simulink library "ammclib_bam_S32K3xx"  (R2016a)
settings: Solver=VariableStepAuto  SolverMode=SingleTasking  StartTime=0.0  StopTime=10.0  RelTol=1e-3
undefined symbols (not defined in the file or in its folder): a1, a2, ADCMaxError, autoCalcEn, b0, b1, b2, cfg, dgain, escale, f16A1, f16A2, f16ADCMaxError, f16B0, f16B1, f16B2, f16C1, f16CC1sc, f16CC1sc_D, f16CC1sc_Q, f16CC2sc, f16CC2sc_D, f16CC2sc_Q, f16DerivGain, f16EGain, f16FiltCoef, f16HystOff, f16HystOn, f16IGain, f16IntegGain, f16IntegGain_D, f16IntegGain_Q, f16IntegGainQ, f16Kd, f16KLs, f16Kq, f16KRs, f16Limit, f16LowerLimit, f16LowerLimit_D, f16LowerLimit_Q, f16LowerLimitQ, f16ModIndex, f16OutValOff, f16OutValOn, f16PropGain, f16PropGain_D, f16PropGain_Q, f16PropGainQ, f16RampDown, f16RampUp, f16UGain, f16UpperLimit, f16UpperLimit_D, f16UpperLimit_Q, f16UpperLimitQ, f16WIGain, f32A1, f32A2, f32ADCMaxError ... (+180)
(part 35 of 50)

== system ammclib_bam_S32K3xx/GFLIB/F32 ==
  GFLIB_Acos_F32 : Subsystem  TreatAsAtomicUnit=on  mask(GFLIB_Acos_F32){}
      mask help: Inverse cosine function in 32-bit fixed-point fractional implementation. Refer to the AMMCLIB User's Guide for further details.
      mask init: same as ammclib_bam_S32K3xx/GDFLIB/F16/GDFLIB_FilterFIR_F16
      settings: RTWSystemCode=Inline
      mask Help: web([fileparts(which('ammclib_bam_S32K3xx.slx')) '/../doc/S32K3XXMCLUG.pdf'], '-browser')
      mask Display: pos = get_param(gcb, 'Position');width = pos(3) - pos(1); height = pos(4) - pos(2);tX=width/2;tY=height - 8;color('black');text(tX,tY, 'GFLIB_Acos_F32', 'horizontalAlignment', 'center');
  GFLIB_Asin_F32 : Subsystem  TreatAsAtomicUnit=on  mask(GFLIB_Asin_F32){}
      mask help: Inverse sine function in 32-bit fixed-point fractional implementation. Refer to the AMMCLIB User's Guide for further details.
      mask init: same as ammclib_bam_S32K3xx/GDFLIB/F16/GDFLIB_FilterFIR_F16
      settings: RTWSystemCode=Inline
      mask Help: web([fileparts(which('ammclib_bam_S32K3xx.slx')) '/../doc/S32K3XXMCLUG.pdf'], '-browser')
      mask Display: pos = get_param(gcb, 'Position');width = pos(3) - pos(1); height = pos(4) - pos(2);tX=width/2;tY=height - 8;color('black');text(tX,tY, 'GFLIB_Asin_F32', 'horizontalAlignment', 'center');
  GFLIB_AtanYXShifted_F32 : Subsystem  TreatAsAtomicUnit=on  mask(GFLIB_AtanYXShifted_F32){}
      mask help: Shifted arctangent of two arguments Y/X in 32-bit fixed-point fractional implementation. Refer to the AMMCLIB User's Guide for further details.
      mask init: same as ammclib_bam_S32K3xx/GDFLIB/F16/GDFLIB_FilterFIR_F16
      settings: RTWSystemCode=Inline
      mask Help: web([fileparts(which('ammclib_bam_S32K3xx.slx')) '/../doc/S32K3XXMCLUG.pdf'], '-browser')
      mask Display: pos = get_param(gcb, 'Position');width = pos(3) - pos(1); height = pos(4) - pos(2);tX=width/2;tY=height - 8;color('black');text(tX,tY, 'GFLIB_AtanYXShifted_F32', 'horizontalAlignment', 'center');
  GFLIB_AtanYX_F32 : Subsystem  TreatAsAtomicUnit=on  mask(GFLIB_AtanYX_F32){}
      mask help: Arctangent of two arguments Y/X in 32-bit fixed-point fractional implementation. Refer to the AMMCLIB User's Guide for further details.
      mask init: same as ammclib_bam_S32K3xx/GDFLIB/F16/GDFLIB_FilterFIR_F16
      settings: RTWSystemCode=Inline
      mask Help: web([fileparts(which('ammclib_bam_S32K3xx.slx')) '/../doc/S32K3XXMCLUG.pdf'], '-browser')
      mask Display: pos = get_param(gcb, 'Position');width = pos(3) - pos(1); height = pos(4) - pos(2);tX=width/2;tY=height - 8;color('black');text(tX,tY, 'GFLIB_AtanYX_F32', 'horizontalAlignment', 'center');
  GFLIB_Atan_F32 : Subsystem  TreatAsAtomicUnit=on  mask(GFLIB_Atan_F32){}
      mask help: Inverse tangent function in 32-bit fixed-point fractional implementation. Refer to the AMMCLIB User's Guide for further details.
      mask init: same as ammclib_bam_S32K3xx/GDFLIB/F16/GDFLIB_FilterFIR_F16
      settings: RTWSystemCode=Inline
      mask Help: web([fileparts(which('ammclib_bam_S32K3xx.slx')) '/../doc/S32K3XXMCLUG.pdf'], '-browser')
      mask Display: pos = get_param(gcb, 'Position');width = pos(3) - pos(1); height = pos(4) - pos(2);tX=width/2;tY=height - 8;color('black');text(tX,tY, 'GFLIB_Atan_F32', 'horizontalAlignment', 'center');
  GFLIB_ControllerPIDpAW_F32 : Subsystem  StartFcn=|  TreatAsAtomicUnit=on  mask(GFLIB_ControllerPIDpAW_F32){showStates=Hide (faster execution), resetStatesEnable=Pre-set according to the first set of inputs after reset, SampleTime=-1, pgain=5, igain=0.5, dgain=0.01, filtCoef=10, lowerLimit=-10, upperLimit=9.999999995343387, inscale=10, outscale=10, autoCalcEn=on, f32PropGain=0, f32IntegGain=0, f32DerivGain=0, f32FiltCoef=0, s16PropGainShift=0, s16IntegGainShift=0, s16DerivGainShift=0, f32LowerLimit=0, f32UpperLimit=0, SampleTime_1=NaN}
      | ts=get_param(gcb,'CompiledSampleTime');
      | if iscell(ts)
      |   ts=ts{1};
      |   if iscell(ts)
      |     ts=ts{1};
      |   end
      | end
      | ts=ts(1);
      | set_param(gcb,'SampleTime_1',num2str(ts));
      | p=Simulink.Mask.get(gcb);
      | hintText=p.getDialogControl('timeHint');
      | SampleTime=Simulink.data.evalinGlobal(bdroot,get_param(gcb,'SampleTime'));
      | p=Simulink.Mask.get(gcb);
      | autoCalcEn=get_param(gcb,'autoCalcEn');
      | if strcmp(autoCalcEn,'on')
      |   if SampleTime==-1
      |     hintText.Prompt='Caution: Implementation parameters depend on inherited sample time. Make sure that the sample time of the block''s inputs corresponds to the sampling period in the target application.';
      |   else
      |     hintText.Prompt='Caution: Implementation parameters depend on the sample time. Make sure that the simulation time step corresponds to the sampling period in the target application.';
      |   end
      |   SampleTime=ts;
      |   f32PropGain_bkup=get_param(gcb,'f32PropGain');
      |   f32IntegGain_bkup=get_param(gcb,'f32IntegGain');
      |   f32DerivGain_bkup=get_param(gcb,'f32DerivGain');
      |   f32FiltCoef_bkup=get_param(gcb,'f32FiltCoef');
      |   s16PropGainShift_bkup=get_param(gcb,'s16PropGainShift');
      |   s16IntegGainShift_bkup=get_param(gcb,'s16IntegGainShift');
      |   s16DerivGainShift_bkup=get_param(gcb,'s16DerivGainShift');
      |   f32LowerLimit_bkup=get_param(gcb,'f32LowerLimit');
      |   f32UpperLimit_bkup=get_param(gcb,'f32UpperLimit');
      |   pgain=Simulink.data.evalinGlobal(bdroot,get_param(gcb,'pgain'));
      |   igain=Simulink.data.evalinGlobal(bdroot,get_param(gcb,'igain'));
      |   dgain=Simulink.data.evalinGlobal(bdroot,get_param(gcb,'dgain'));
      |   filtCoef=Simulink.data.evalinGlobal(bdroot,get_param(gcb,'filtCoef'));
      |   lowerLimit=Simulink.data.evalinGlobal(bdroot,get_param(gcb,'lowerLimit'));
      |   upperLimit=Simulink.data.evalinGlobal(bdroot,get_param(gcb,'upperLimit'));
      |   inscale=Simulink.data.evalinGlobal(bdroot,get_param(gcb,'inscale'));
      |   outscale=Simulink.data.evalinGlobal(bdroot,get_param(gcb,'outscale'));
      |   if (upperLimit<=lowerLimit)
      |     warning('UpperLimit should be greater than LowerLimit.');
      |   end
      |   if (inscale<=0)
      |     warning('E_max must be positive.');
      |   end
      |   if (outscale<=0)
      |     warning('U_max must be positive.');
      |   end
      |   kpf=pgain*inscale/outscale;
      |   s16PropGainShift=ceil(log2(abs(kpf)));
      |   if s16PropGainShift<-31
      |     s16PropGainShift=-31;
      |   end
      |   if s16PropGainShift>31
      |     s16PropGainShift=31;
      |     warning(['Parameter s16PropGainShift of ' gcb ' exceeds the fixed-point range.']);
      |   end
      |   f32PropGain=round(kpf*2^(-s16PropGainShift)*2^31);
      |   if f32PropGain>2^31-1
      |     f32PropGain=2^31-1;
      |     warning(['Parameter f32PropGain of ' gcb ' exceeds the fixed-point range.']);
      |   end
      |   if f32PropGain<-2^31
      |     f32PropGain=-2^31;
      |     warning(['Parameter f32PropGain of ' gcb ' exceeds the fixed-point range.']);
      |   end
      |   kif=igain*SampleTime*0.5*inscale/outscale;
      |   s16IntegGainShift=ceil(log2(abs(kif)));
      |   if s16IntegGainShift<-31
      |     s16IntegGainShift=-31;
      |   end
      |   if s16IntegGainShift>31
      |     s16IntegGainShift=31;
      |     warning(['Parameter s16IntegGainShift of ' gcb ' exceeds the fixed-point range.']);
      |   end
      |   f32IntegGain=round(kif*2^(-s16IntegGainShift)*2^31);
      |   if f32IntegGain>2^31-1
      |     f32IntegGain=2^31-1;
      |     warning(['Parameter f32IntegGain of ' gcb ' exceeds the fixed-point range.']);
      |   end
      |   if f32IntegGain<-2^31
      |     f32IntegGain=-2^31;
      |     warning(['Parameter f32IntegGain of ' gcb ' exceeds the fixed-point range.']);
      |   end
      |   upperLimitf=upperLimit/outscale;
      |   lowerLimitf=lowerLimit/outscale;
      |   f32UpperLimit=round(upperLimitf*2^31);
      |   if f32UpperLimit>2^31-1
      |     f32UpperLimit=2^31-1;
      |     warning(['Parameter f32UpperLimit of ' gcb ' exceeds the fixed-point range.']);
      |   end
      |   if f32UpperLimit<-2^31
      |     f32UpperLimit=-2^31;
      |     warning(['Parameter f32UpperLimit of ' gcb ' exceeds the fixed-point range.']);
      |   end
      |   f32LowerLimit=round(lowerLimitf*2^31);
      |   if f32LowerLimit>2^31-1
      |     f32LowerLimit=2^31-1;
      |     warning(['Parameter f32LowerLimit of ' gcb ' exceeds the fixed-point range.']);
      |   end
      |   if f32LowerLimit<-2^31
      |     f32LowerLimit=-2^31;
      |     warning(['Parameter f32LowerLimit of ' gcb ' exceeds the fixed-point range.']);
      |   end
      |   exparg=-SampleTime*filtCoef;
      |   expconst=exp(exparg);
      |   f32FiltCoef=round(expconst*2^31);
      |   if f32FiltCoef>2^31-1
      |     f32FiltCoef=2^31-1;
      |     warning(['Parameter f32FiltCoef of ' gcb ' exceeds the fixed-point range.']);
      |   end
      |   if f32FiltCoef<-2^31
      |     f32FiltCoef=-2^31;
      |     warning(['Parameter f32FiltCoef of ' gcb ' exceeds the fixed-point range.']);
      |   end
      |   kdf=dgain/SampleTime*(1 - expconst)*inscale/outscale;
      |   s16DerivGainShift=ceil(log2(abs(kpf)));
      |   if s16DerivGainShift<-31
      |     s16DerivGainShift=-31;
      |   end
      |   if s16DerivGainShift>31
      |     s16DerivGainShift=31;
      |     warning(['Parameter s16DerivGainShift of ' gcb ' exceeds the fixed-point range.']);
      |   end
      |   f32DerivGain=round(kpf*2^(-s16DerivGainShift)*2^31);
      |   if f32DerivGain>2^31-1
      |     f32DerivGain=2^31-1;
      |     warning(['Parameter f32DerivGain of ' gcb ' exceeds the fixed-point range.']);
      |   end
      |   if f32DerivGain<-2^31
      |     f32DerivGain=-2^31;
      |     warning(['Parameter f32DerivGain of ' gcb ' exceeds the fixed-point range.']);
      |   end
      |   if isnan(f32PropGain)
      |     if ~strcmp(f32PropGain_bkup,'0')
      |       set_param(gcb,'f32PropGain','0');
      |     end
      |   else
      |     tmps=num2str(f32PropGain);
      |     if ~strcmp(f32PropGain_bkup,tmps)
      |       set_param(gcb,'f32PropGain',tmps);
      |     end
      |   end
      |   if isnan(f32IntegGain)
      |     if ~strcmp(f32IntegGain_bkup,'0')
      |       set_param(gcb,'f32IntegGain','0');
      |     end
      |   else
      |     tmps=num2str(f32IntegGain);
      |     if ~strcmp(f32IntegGain_bkup,tmps)
      |       set_param(gcb,'f32IntegGain',tmps);
      |     end
      |   end
      |   if isnan(f32DerivGain)
      |     if ~strcmp(f32DerivGain_bkup,'0')
      |       set_param(gcb,'f32DerivGain','0');
      |     end
      |   else
      |     tmps=num2str(f32DerivGain);
      |     if ~strcmp(f32DerivGain_bkup,tmps)
      |       set_param(gcb,'f32DerivGain',tmps);
      |     end
      |   end
      |   if isnan(f32FiltCoef)
      |     if ~strcmp(f32FiltCoef_bkup,'0')
      |       set_param(gcb,'f32FiltCoef','0');
      |     end
      |   else
      |     tmps=num2str(f32FiltCoef);
      |     if ~strcmp(f32FiltCoef_bkup,tmps)
      |       set_param(gcb,'f32FiltCoef',tmps);
      |     end
      |   end
      |   if isnan(s16PropGainShift)
      |     if ~strcmp(s16PropGainShift_bkup,'0')
      |       set_param(gcb,'s16PropGainShift','0');
      |     end
      |   else
      |     tmps=num2str(s16PropGainShift);
      |     if ~strcmp(s16PropGainShift_bkup,tmps)
      |       set_param(gcb,'s16PropGainShift',tmps);
      |     end
      |   end
      |   if isnan(s16IntegGainShift)
      |     if ~strcmp(s16IntegGainShift_bkup,'0')
      |       set_param(gcb,'s16IntegGainShift','0');
      |     end
      |   else
      |     tmps=num2str(s16IntegGainShift);
      |     if ~strcmp(s16IntegGainShift_bkup,tmps)
      |       set_param(gcb,'s16IntegGainShift',tmps);
      |     end
      |   end
      |   if isnan(s16DerivGainShift)
      |     if ~strcmp(s16DerivGainShift_bkup,'0')
      |       set_param(gcb,'s16DerivGainShift','0');
      |     end
      |   else
      |     tmps=num2str(s16DerivGainShift);
      |     if ~strcmp(s16DerivGainShift_bkup,tmps)
      |       set_param(gcb,'s16DerivGainShift',tmps);
      |     end
      |   end
      |   if isnan(f32LowerLimit)
      |     if ~strcmp(f32LowerLimit_bkup,'0')
      |       set_param(gcb,'f32LowerLimit','0');
      |     end
      |   else
      |     tmps=num2str(f32LowerLimit);
      |     if ~strcmp(f32LowerLimit_bkup,tmps)
      |       set_param(gcb,'f32LowerLimit',tmps);
      |     end
      |   end
      |   if isnan(f32UpperLimit)
      |     if ~strcmp(f32UpperLimit_bkup,'0')
      |       set_param(gcb,'f32UpperLimit','0');
      |     end
      |   else
      |     tmps=num2str(f32UpperLimit);
      |     if ~strcmp(f32UpperLimit_bkup,tmps)
      |       set_param(gcb,'f32UpperLimit',tmps);
      |     end
      |   end
      | end
      mask prompts: showStates "Show internal states:"; resetStatesEnable "Internal state after reset:"; SampleTime "Sample time (-1 for inherited):"; pgain "Proportional gain (P):"; igain "Integral gain (I):"; dgain "Derivative gain (D):"; filtCoef "Derivative gain limit N (usually 3 to 20):"; lowerLimit "Controller lower limit:"; upperLimit "Controller upper limit:"; inscale "E_max (input scale):"; outscale "U_max (output scale):"; autoCalcEn "Calculate implementation parameters from physical parameters"; f32PropGain "f32PropGain (Proportional gain):"; f32IntegGain "f32IntegGain (Integral gain):"; f32DerivGain "f32DerivGain (Derivative gain):"; f32FiltCoef "f32FiltCoef (Derivative term filter coefficient):"; s16PropGainShift "s16PropGainShift (Proportional gain shift):"; s16IntegGainShift "s16IntegGainShift (Integral gain shift):"; s16DerivGainShift "s16DerivGainShift (Derivative gain shift):"; f32LowerLimit "f32LowerLimit (Lower limit of the controller):"; f32UpperLimit "f32UpperLimit (Upper limit of the controller):"; SampleTime_1 "Discrete sample time:"
      mask help: Parallel form of a discrete-time PID controller with anti-windup in 32-bit fixed-point fractional implementation. This block supports re-initialization of the internal state during simulation. If the block is reset, the controller's output will be aligned with the input f32ControllerPIDpAWOut_preset. Refer to the AMMCLIB User's Guide for further details.
      mask init:
      | ddName = get_param(bdroot,'DataDictionary');
      | if length(ddName)==0
      |   set_param(bdroot,'DataDictionary','ammclib_types.sldd');
      | else
      |   dd = Simulink.data.dictionary.open(ddName);
      |   data = getSection(dd,'Design Data');
      |   if ~exist(data,'SWLIBS_2Syst_F16')
      |     addDataSource(dd,'ammclib_types.sldd');
      |     saveChanges(dd);
      |   end
      | end
      | 
      | if showStates == 1
      |   % hidden state variables
      |   if strcmp(get_param([gcb '/f32PropGain'], 'BlockType'), 'Inport')
      |     posblk = get_param(gcb, 'Position');
      | 
      |     pos = get_param([gcb, '/f32PropGain'], 'Position');
      |     orient = get_param([gcb, '/f32PropGain'], 'Orientation');
      |     delete_block([gcb, '/f32PropGain']);
      |     add_block('built-in/Ground', [gcb, '/f32PropGain'], 'Position', pos, 'Orientation', orient);
      | 
      |     pos = get_param([gcb, '/f32IntegGain'], 'Position');
      |     orient = get_param([gcb, '/f32IntegGain'], 'Orientation');
      |     delete_block([gcb, '/f32IntegGain']);
      |     add_block('built-in/Ground', [gcb, '/f32IntegGain'], 'Position', pos, 'Orientation', orient);
      | 
      |     pos = get_param([gcb, '/f32DerivGain'], 'Position');
      |     orient = get_param([gcb, '/f32DerivGain'], 'Orientation');
      |     delete_block([gcb, '/f32DerivGain']);
      |     add_block('built-in/Ground', [gcb, '/f32DerivGain'], 'Position', pos, 'Orientation', orient);
      | 
      |     pos = get_param([gcb, '/f32FiltCoef'], 'Position');
      |     orient = get_param([gcb, '/f32FiltCoef'], 'Orientation');
      |     delete_block([gcb, '/f32FiltCoef']);
      |     add_block('built-in/Ground', [gcb, '/f32FiltCoef'], 'Position', pos, 'Orientation', orient);
      | 
      |     pos = get_param([gcb, '/s16PropGainShift'], 'Position');
      |     orient = get_param([gcb, '/s16PropGainShift'], 'Orientation');
      |     delete_block([gcb, '/s16PropGainShift']);
      |     add_block('built-in/Ground', [gcb, '/s16PropGainShift'], 'Position', pos, 'Orientation', orient);
      | 
      |     pos = get_param([gcb, '/s16IntegGainShift'], 'Position');
      |     orient = get_param([gcb, '/s16IntegGainShift'], 'Orientation');
      |     delete_block([gcb, '/s16IntegGainShift']);
      |     add_block('built-in/Ground', [gcb, '/s16IntegGainShift'], 'Position', pos, 'Orientation', orient);
      | 
      |     pos = get_param([gcb, '/s16DerivGainShift'], 'Position');
      |     orient = get_param([gcb, '/s16DerivGainShift'], 'Orientation');
      |     delete_block([gcb, '/s16DerivGainShift']);
      |     add_block('built-in/Ground', [gcb, '/s16DerivGainShift'], 'Position', pos, 'Orientation', orient);
      | 
      |     pos = get_param([gcb, '/f32LowerLimit'], 'Position');
      |     orient = get_param([gcb, '/f32LowerLimit'], 'Orientation');
      |     delete_block([gcb, '/f32LowerLimit']);
      |     add_block('built-in/Ground', [gcb, '/f32LowerLimit'], 'Position', pos, 'Orientation', orient);
      | 
      |     pos = get_param([gcb, '/f32UpperLimit'], 'Position');
      |     orient = get_param([gcb, '/f32UpperLimit'], 'Orientation');
      |     delete_block([gcb, '/f32UpperLimit']);
      |     add_block('built-in/Ground', [gcb, '/f32UpperLimit'], 'Position', pos, 'Orientation', orient);
      | 
      |     pos = get_param([gcb, '/f32IntegPartK_1'], 'Position');
      |     orient = get_param([gcb, '/f32IntegPartK_1'], 'Orientation');
      |     delete_block([gcb, '/f32IntegPartK_1']);
      |     add_block('built-in/Ground', [gcb, '/f32IntegPartK_1'], 'Position', pos, 'Orientation', orient);
      | 
      |     pos = get_param([gcb, '/f32DerivPartK_1'], 'Position');
      |     orient = get_param([gcb, '/f32DerivPartK_1'], 'Orientation');
      |     delete_block([gcb, '/f32DerivPartK_1']);
      |     add_block('built-in/Ground', [gcb, '/f32DerivPartK_1'], 'Position', pos, 'Orientation', orient);
      | 
      |     pos = get_param([gcb, '/f32InK_1'], 'Position');
      |     orient = get_param([gcb, '/f32InK_1'], 'Orientation');
      |     delete_block([gcb, '/f32InK_1']);
      |     add_block('built-in/Ground', [gcb, '/f32InK_1'], 'Position', pos, 'Orientation', orient);
      | 
      | 
      |     pmask=Simulink.Mask.get(gcb);
      |     pctrl=pmask.getParameter('SampleTime');
      |     pctrl.set('TypeOptions',{'f32InErr/SampleTime','f32ControllerPIDpAWOut_preset/SampleTime'});
      | 
      |     pos = get_param([gcb '/f32IntegPartK_1_Out'], 'Position');
      |     orient = get_param([gcb '/f32IntegPartK_1_Out'], 'Orientation');
      |     delete_block([gcb '/f32IntegPartK_1_Out']);
      |     add_block('built-in/Terminator', [gcb '/f32IntegPartK_1_Out'], 'Position', pos, 'Orientation', orient);
      | 
      |     pos = get_param([gcb '/f32DerivPartK_1_Out'], 'Position');
      |     orient = get_param([gcb '/f32DerivPartK_1_Out'], 'Orientation');
      |     delete_block([gcb '/f32DerivPartK_1_Out']);
      |     add_block('built-in/Terminator', [gcb '/f32DerivPartK_1_Out'], 'Position', pos, 'Orientation', orient);
      | 
      |     pos = get_param([gcb '/f32InK_1_Out'], 'Position');
      |     orient = get_param([gcb '/f32InK_1_Out'], 'Orientation');
      |     delete_block([gcb '/f32InK_1_Out']);
      |     add_block('built-in/Terminator', [gcb '/f32InK_1_Out'], 'Position', pos, 'Orientation', orient);
      | 
      |     set_param([gcb '/f32InErr'], 'Port', '1');
      |     set_param([gcb '/f32ControllerPIDpAWOut_preset'], 'Port', '2');
      | 
      |     tmpOutCnt=0;
      |     tmpOutCnt=tmpOutCnt+1;
      |     set_param([gcb '/f32Out'], 'Port', num2str(tmpOutCnt));
      |     tmpOutCnt=tmpOutCnt+1;
      |     set_param([gcb '/u16LimitFlag'], 'Port', num2str(tmpOutCnt));
      | 
      |     autoCalcEn=get_param(gcb,'autoCalcEn');
      |     if strcmp(autoCalcEn,'on')
      |       set_param(gcb,'MaskEnables',{'on','on','on','on','on','on','on','on','on','on','on','on','on','on','on','on','on','on','on','on','on','off'});
      |     else
      |       set_param(gcb,'MaskEnables',{'on','on','on','off','off','off','off','off','off','off','off','on','on','on','on','on','on','on','on','on','on','off'});
      |     end
      | 
      |     if (posblk(4) - posblk(2)) > 75
      |       height = 75;
      |       set_param(gcb,'Position',[posblk(1), posblk(2), posblk(3), posblk(2)+height])
      |     end
      |   end
      | else
      |   % shown state variables
      |   if strcmp(get_param([gcb '/f32PropGain'], 'BlockType'), 'Ground')
      |     posblk = get_param(gcb, 'Position');
      | 
      |     pos = get_param([gcb, '/f32PropGain'], 'Position');
      |     orient = get_param([gcb, '/f32PropGain'], 'Orientation');
      |     delete_block([gcb, '/f32PropGain']);
      |     add_block('built-in/Inport', [gcb, '/f32PropGain'], 'Position', pos, 'Orientation', orient, 'OutDataTypeStr', 'int32');
      | 
      |     pos = get_param([gcb, '/f32IntegGain'], 'Position');
      |     orient = get_param([gcb, '/f32IntegGain'], 'Orientation');
      |     delete_block([gcb, '/f32IntegGain']);
      |     add_block('built-in/Inport', [gcb, '/f32IntegGain'], 'Position', pos, 'Orientation', orient, 'OutDataTypeStr', 'int32');
      | 
      |     pos = get_param([gcb, '/f32DerivGain'], 'Position');
      |     orient = get_param([gcb, '/f32DerivGain'], 'Orientation');
      |     delete_block([gcb, '/f32DerivGain']);
      |     add_block('built-in/Inport', [gcb, '/f32DerivGain'], 'Position', pos, 'Orientation', orient, 'OutDataTypeStr', 'int32');
      | 
      |     pos = get_param([gcb, '/f32FiltCoef'], 'Position');
      |     orient = get_param([gcb, '/f32FiltCoef'], 'Orientation');
      |     delete_block([gcb, '/f32FiltCoef']);
      |     add_block('built-in/Inport', [gcb, '/f32FiltCoef'], 'Position', pos, 'Orientation', orient, 'OutDataTypeStr', 'int32');
      | 
      |     pos = get_param([gcb, '/s16PropGainShift'], 'Position');
      |     orient = get_param([gcb, '/s16PropGainShift'], 'Orientation');
      |     delete_block([gcb, '/s16PropGainShift']);
      |     add_block('built-in/Inport', [gcb, '/s16PropGainShift'], 'Position', pos, 'Orientation', orient, 'OutDataTypeStr', 'int16');
      | 
      |     pos = get_param([gcb, '/s16IntegGainShift'], 'Position');
      |     orient = get_param([gcb, '/s16IntegGainShift'], 'Orientation');
      |     delete_block([gcb, '/s16IntegGainShift']);
      |     add_block('built-in/Inport', [gcb, '/s16IntegGainShift'], 'Position', pos, 'Orientation', orient, 'OutDataTypeStr', 'int16');
      | 
      |     pos = get_param([gcb, '/s16DerivGainShift'], 'Position');
      |     orient = get_param([gcb, '/s16DerivGainShift'], 'Orientation');
      |     delete_block([gcb, '/s16DerivGainShift']);
      |     add_block('built-in/Inport', [gcb, '/s16DerivGainShift'], 'Position', pos, 'Orientation', orient, 'OutDataTypeStr', 'int16');
      | 
      |     pos = get_param([gcb, '/f32LowerLimit'], 'Position');
      |     orient = get_param([gcb, '/f32LowerLimit'], 'Orientation');
      |     delete_block([gcb, '/f32LowerLimit']);
      |     add_block('built-in/Inport', [gcb, '/f32LowerLimit'], 'Position', pos, 'Orientation', orient, 'OutDataTypeStr', 'int32');
      | 
      |     pos = get_param([gcb, '/f32UpperLimit'], 'Position');
      |     orient = get_param([gcb, '/f32UpperLimit'], 'Orientation');
      |     delete_block([gcb, '/f32UpperLimit']);
      |     add_block('built-in/Inport', [gcb, '/f32UpperLimit'], 'Position', pos, 'Orientation', orient, 'OutDataTypeStr', 'int32');
      | 
      |     pos = get_param([gcb, '/f32IntegPartK_1'], 'Position');
      |     orient = get_param([gcb, '/f32IntegPartK_1'], 'Orientation');
      |     delete_block([gcb, '/f32IntegPartK_1']);
      |     add_block('built-in/Inport', [gcb, '/f32IntegPartK_1'], 'Position', pos, 'Orientation', orient, 'OutDataTypeStr', 'int32');
      | 
      |     pos = get_param([gcb, '/f32DerivPartK_1'], 'Position');
      |     orient = get_param([gcb, '/f32DerivPartK_1'], 'Orientation');
      |     delete_block([gcb, '/f32DerivPartK_1']);
      |     add_block('built-in/Inport', [gcb, '/f32DerivPartK_1'], 'Position', pos, 'Orientation', orient, 'OutDataTypeStr', 'int32');
      | 
      |     pos = get_param([gcb, '/f32InK_1'], 'Position');
      |     orient = get_param([gcb, '/f32InK_1'], 'Orientation');
      |     delete_block([gcb, '/f32InK_1']);
      |     add_block('built-in/Inport', [gcb, '/f32InK_1'], 'Position', pos, 'Orientation', orient, 'OutDataTypeStr', 'int32');
      | 
      | 
      | 
      |     pos = get_param([gcb '/f32IntegPartK_1_Out'], 'Position');
      |     orient = get_param([gcb '/f32IntegPartK_1_Out'], 'Orientation');
      |     delete_block([gcb '/f32IntegPartK_1_Out']);
      |     add_block('built-in/Outport', [gcb '/f32IntegPartK_1_Out'], 'Position', pos, 'Orientation', orient);
      | 
      |     pos = get_param([gcb '/f32DerivPartK_1_Out'], 'Position');
      |     orient = get_param([gcb '/f32DerivPartK_1_Out'], 'Orientation');
      |     delete_block([gcb '/f32DerivPartK_1_Out']);
      |     add_block('built-in/Outport', [gcb '/f32DerivPartK_1_Out'], 'Position', pos, 'Orientation', orient);
      | 
      |     pos = get_param([gcb '/f32InK_1_Out'], 'Position');
      |     orient = get_param([gcb '/f32InK_1_Out'], 'Orientation');
      |     delete_block([gcb '/f32InK_1_Out']);
      |     add_block('built-in/Outport', [gcb '/f32InK_1_Out'], 'Position', pos, 'Orientation', orient);
      | 
      | 
      |     pmask=Simulink.Mask.get(gcb);
      |     pctrl=pmask.getParameter('SampleTime');
      |     pctrl.set('TypeOptions',{'f32InErr/SampleTime','f32ControllerPIDpAWOut_preset/SampleTime','f32PropGain/SampleTime','f32IntegGain/SampleTime','f32DerivGain/SampleTime','f32FiltCoef/SampleTime','s16PropGainShift/SampleTime','s16IntegGainShift/SampleTime','s16DerivGainShift/SampleTime','f32LowerLimit/SampleTime','f32UpperLimit/SampleTime','f32IntegPartK_1/SampleTime','f32DerivPartK_1/SampleTime','f32InK_1/SampleTime'});
      | 
      |     set_param([gcb '/f32InErr'], 'Port', '1');
      |     set_param([gcb '/f32ControllerPIDpAWOut_preset'], 'Port', '2');
      |     set_param([gcb '/f32PropGain'], 'Port', '3');
      |     set_param([gcb '/f32IntegGain'], 'Port', '4');
      |     set_param([gcb '/f32DerivGain'], 'Port', '5');
      |     set_param([gcb '/f32FiltCoef'], 'Port', '6');
      |     set_param([gcb '/s16PropGainShift'], 'Port', '7');
      |     set_param([gcb '/s16IntegGainShift'], 'Port', '8');
      |     set_param([gcb '/s16DerivGainShift'], 'Port', '9');
      |     set_param([gcb '/f32LowerLimit'], 'Port', '10');
      |     set_param([gcb '/f32UpperLimit'], 'Port', '11');
      |     set_param([gcb '/f32IntegPartK_1'], 'Port', '12');
      |     set_param([gcb '/f32DerivPartK_1'], 'Port', '13');
      |     set_param([gcb '/f32InK_1'], 'Port', '14');
      | 
      |     tmpOutCnt=0;
      |     tmpOutCnt=tmpOutCnt+1;
      |     set_param([gcb '/f32Out'], 'Port', num2str(tmpOutCnt));
      |     tmpOutCnt=tmpOutCnt+1;
      |     set_param([gcb '/u16LimitFlag'], 'Port', num2str(tmpOutCnt));
      |     tmpOutCnt=tmpOutCnt+1;
      |     set_param([gcb '/f32IntegPartK_1_Out'], 'Port', num2str(tmpOutCnt));
      |     tmpOutCnt=tmpOutCnt+1;
      |     set_param([gcb '/f32DerivPartK_1_Out'], 'Port', num2str(tmpOutCnt));
      |     tmpOutCnt=tmpOutCnt+1;
      |     set_param([gcb '/f32InK_1_Out'], 'Port', num2str(tmpOutCnt));
      | 
      |     set_param(gcb,'MaskEnables',{'on','on','on','off','off','off','off','off','off','off','off','off','off','off','off','off','off','off','off','off','off','off'});
      | 
      |     if (posblk(4) - posblk(2)) < 375
      |       height = 375;
      |       set_param(gcb,'Position',[posblk(1), posblk(2), posblk(3), posblk(2)+height])
      |     end
      |   end
      | end
      settings: RTWSystemCode=Inline
      mask Help: web([fileparts(which('ammclib_bam_S32K3xx.slx')) '/../doc/S32K3XXMCLUG.pdf'], '-browser')
      mask TypeOptions showStates: Hide (faster execution) | Show (allows debugging; connect feedback loops manually)
      mask Callback showStates:
      | maskStr=get_param(gcb,'showStates');
      | if strcmp(maskStr,'Hide (faster execution)')
      |   if strcmp(get_param([gcb '/f32PropGain'], 'BlockType'), 'Inport')
      |     autoCalcEn=get_param(gcb,'autoCalcEn');
      |     if strcmp(autoCalcEn,'on')
      |       set_param(gcb,'MaskEnables',{'on','on','on','on','on','on','on','on','on','on','on','on','on','on','on','on','on','on','on','on','on','off'});
      |     else
      |       set_param(gcb,'MaskEnables',{'on','on','on','off','off','off','off','off','off','off','off','on','on','on','on','on','on','on','on','on','on','off'});
      |     end
      |   end
      | else
      |   if strcmp(get_param([gcb '/f32PropGain'], 'BlockType'), 'Ground')
      |     set_param(gcb,'MaskEnables',{'on','on','on','off','off','off','off','off','off','off','off','off','off','off','off','off','off','off','off','off','off','off'});
      |   end
      | end
      mask TypeOptions resetStatesEnable: Pre-set according to the first set of inputs after reset | Clear to zero
      mask TypeOptions SampleTime: f32InErr/SampleTime | f32ControllerPIDpAWOut_preset/SampleTime
      mask Callback SampleTime:
      | p=Simulink.Mask.get(gcb);
      | hintText=p.getDialogControl('timeHint');
      | SampleTime=Simulink.data.evalinGlobal(bdroot,get_param(gcb,'SampleTime'));
      | SampleTime_1=str2double(get_param(gcb,'SampleTime_1'));
      | if (((SampleTime==-1) && (~contains(hintText.Prompt,'inherited'))) || ...
      |     ((SampleTime~=-1) && contains(hintText.Prompt,'inherited')) || ...
      |     ((SampleTime~=-1) && (SampleTime_1~=SampleTime)) || ...
      |     ((SampleTime_1~=-1) && contains(hintText.Prompt,'yet')))
      |   if ((SampleTime==-1) && (~contains(hintText.Prompt,'inherited')))
      |     set_param(gcb,'SampleTime_1',num2str(NaN));
      |     SampleTime_1=NaN;
      |   end
      |   if (SampleTime~=-1)
      |     set_param(gcb,'SampleTime_1',num2str(SampleTime));
      |     SampleTime_1=SampleTime;
      |   end
      |   autoCalcEn=get_param(gcb,'autoCalcEn');
      |   if strcmp(autoCalcEn,'on')
      |     p=Simulink.Mask.get(gcb);
      |     hintText=p.getDialogControl('timeHint');
      |     if SampleTime==-1
      |       SampleTime=SampleTime_1;
      |       if isnan(SampleTime)
      |         hintText.Prompt='Note: Implementation parameters cannot be calculated yet because the block''s inherited sample time is unknown. Simulink will update the sample time when you run the simulation.';
      |       else
      |         hintText.Prompt='Caution: Implementation parameters depend on inherited sample time. Make sure that the sample time of the block''s inputs corresponds to the sampling period in the target application.';
      |       end
      |     else
      |       hintText.Prompt='Caution: Implementation parameters depend on the sample time. Make sure that the simulation time step corresponds to the sampling period in the target application.';
      |     end
      |     f32PropGain_bkup=get_param(gcb,'f32PropGain');
      |     f32IntegGain_bkup=get_param(gcb,'f32IntegGain');
      |     f32DerivGain_bkup=get_param(gcb,'f32DerivGain');
      |     f32FiltCoef_bkup=get_param(gcb,'f32FiltCoef');
      |     s16PropGainShift_bkup=get_param(gcb,'s16PropGainShift');
      |     s16IntegGainShift_bkup=get_param(gcb,'s16IntegGainShift');
      |     s16DerivGainShift_bkup=get_param(gcb,'s16DerivGainShift');
      |     f32LowerLimit_bkup=get_param(gcb,'f32LowerLimit');
      |     f32UpperLimit_bkup=get_param(gcb,'f32UpperLimit');
      |     pgain=Simulink.data.evalinGlobal(bdroot,get_param(gcb,'pgain'));
      |     igain=Simulink.data.evalinGlobal(bdroot,get_param(gcb,'igain'));
      |     dgain=Simulink.data.evalinGlobal(bdroot,get_param(gcb,'dgain'));
      |     filtCoef=Simulink.data.evalinGlobal(bdroot,get_param(gcb,'filtCoef'));
      |     lowerLimit=Simulink.data.evalinGlobal(bdroot,get_param(gcb,'lowerLimit'));
      |     upperLimit=Simulink.data.evalinGlobal(bdroot,get_param(gcb,'upperLimit'));
      |     inscale=Simulink.data.evalinGlobal(bdroot,get_param(gcb,'inscale'));
      |     outscale=Simulink.data.evalinGlobal(bdroot,get_param(gcb,'outscale'));
      |     if (upperLimit<=lowerLimit)
      |       warning('UpperLimit should be greater than LowerLimit.');
      |     end
      |     if (inscale<=0)
      |       warning('E_max must be positive.');
      |     end
      |     if (outscale<=0)
      |       warning('U_max must be positive.');
      |     end
      |     kpf=pgain*inscale/outscale;
      |     s16PropGainShift=ceil(log2(abs(kpf)));
      |     if s16PropGainShift<-31
      |       s16PropGainShift=-31;
      |     end
      |     if s16PropGainShift>31
      |       s16PropGainShift=31;
      |       warning(['Parameter s16PropGainShift of ' gcb ' exceeds the fixed-point range.']);
      |     end
      |     f32PropGain=round(kpf*2^(-s16PropGainShift)*2^31);
      |     if f32PropGain>2^31-1
      |       f32PropGain=2^31-1;
      |       warning(['Parameter f32PropGain of ' gcb ' exceeds the fixed-point range.']);
      |     end
      |     if f32PropGain<-2^31
      |       f32PropGain=-2^31;
      |       warning(['Parameter f32PropGain of ' gcb ' exceeds the fixed-point range.']);
      |     end
      |     kif=igain*SampleTime*0.5*inscale/outscale;
      |     s16IntegGainShift=ceil(log2(abs(kif)));
      |     if s16IntegGainShift<-31
      |       s16IntegGainShift=-31;
      |     end
      |     if s16IntegGainShift>31
      |       s16IntegGainShift=31;
      |       warning(['Parameter s16IntegGainShift of ' gcb ' exceeds the fixed-point range.']);
      |     end
      |     f32IntegGain=round(kif*2^(-s16IntegGainShift)*2^31);
      |     if f32IntegGain>2^31-1
      |       f32IntegGain=2^31-1;
      |       warning(['Parameter f32IntegGain of ' gcb ' exceeds the fixed-point range.']);
      |     end
      |     if f32IntegGain<-2^31
      |       f32IntegGain=-2^31;
      |       warning(['Parameter f32IntegGain of ' gcb ' exceeds the fixed-point range.']);
      |     end
      |     upperLimitf=upperLimit/outscale;
      |     lowerLimitf=lowerLimit/outscale;
      |     f32UpperLimit=round(upperLimitf*2^31);
      |     if f32UpperLimit>2^31-1
      |       f32UpperLimit=2^31-1;
      |       warning(['Parameter f32UpperLimit of ' gcb ' exceeds the fixed-point range.']);
      |     end
      |     if f32UpperLimit<-2^31
      |       f32UpperLimit=-2^31;
      |       warning(['Parameter f32UpperLimit of ' gcb ' exceeds the fixed-point range.']);
      |     end
      |     f32LowerLimit=round(lowerLimitf*2^31);
      |     if f32LowerLimit>2^31-1
      |       f32LowerLimit=2^31-1;
      |       warning(['Parameter f32LowerLimit of ' gcb ' exceeds the fixed-point range.']);
      |     end
      |     if f32LowerLimit<-2^31
      |       f32LowerLimit=-2^31;
      |       warning(['Parameter f32LowerLimit of ' gcb ' exceeds the fixed-point range.']);
      |     end
      |     exparg=-SampleTime*filtCoef;
      |     expconst=exp(exparg);
      |     f32FiltCoef=round(expconst*2^31);
      |     if f32FiltCoef>2^31-1
      |       f32FiltCoef=2^31-1;
      |       warning(['Parameter f32FiltCoef of ' gcb ' exceeds the fixed-point range.']);
      |     end
      |     if f32FiltCoef<-2^31
      |       f32FiltCoef=-2^31;
      |       warning(['Parameter f32FiltCoef of ' gcb ' exceeds the fixed-point range.']);
      |     end
      |     kdf=dgain/SampleTime*(1 - expconst)*inscale/outscale;
      |     s16DerivGainShift=ceil(log2(abs(kpf)));
      |     if s16DerivGainShift<-31
      |       s16DerivGainShift=-31;
      |     end
      |     if s16DerivGainShift>31
      |       s16DerivGainShift=31;
      |       warning(['Parameter s16DerivGainShift of ' gcb ' exceeds the fixed-point range.']);
      |     end
      |     f32DerivGain=round(kpf*2^(-s16DerivGainShift)*2^31);
      |     if f32DerivGain>2^31-1
      |       f32DerivGain=2^31-1;
      |       warning(['Parameter f32DerivGain of ' gcb ' exceeds the fixed-point range.']);
      |     end
      |     if f32DerivGain<-2^31
      |       f32DerivGain=-2^31;
      |       warning(['Parameter f32DerivGain of ' gcb ' exceeds the fixed-point range.']);
      |     end
      |     if isnan(f32PropGain)
      |       if ~strcmp(f32PropGain_bkup,'0')
      |         set_param(gcb,'f32PropGain','0');
      |       end
      |     else
      |       tmps=num2str(f32PropGain);
      |       if ~strcmp(f32PropGain_bkup,tmps)
      |         set_param(gcb,'f32PropGain',tmps);
      |       end
      |     end
      |     if isnan(f32IntegGain)
      |       if ~strcmp(f32IntegGain_bkup,'0')
      |         set_param(gcb,'f32IntegGain','0');
      |       end
      |     else
      |       tmps=num2str(f32IntegGain);
      |       if ~strcmp(f32IntegGain_bkup,tmps)
      |         set_param(gcb,'f32IntegGain',tmps);
      |       end
      |     end
      |     if isnan(f32DerivGain)
      |       if ~strcmp(f32DerivGain_bkup,'0')
      |         set_param(gcb,'f32DerivGain','0');
      |       end
      |     else
      |       tmps=num2str(f32DerivGain);
      |       if ~strcmp(f32DerivGain_bkup,tmps)
      |         set_param(gcb,'f32DerivGain',tmps);
      |       end
      |     end
      |     if isnan(f32FiltCoef)
      |       if ~strcmp(f32FiltCoef_bkup,'0')
      |         set_param(gcb,'f32FiltCoef','0');
      |       end
      |     else
      |       tmps=num2str(f32FiltCoef);
      |       if ~strcmp(f32FiltCoef_bkup,tmps)
      |         set_param(gcb,'f32FiltCoef',tmps);
      |       end
      |     end
      |     if isnan(s16PropGainShift)
      |       if ~strcmp(s16PropGainShift_bkup,'0')
      |         set_param(gcb,'s16PropGainShift','0');
      |       end
      |     else
      |       tmps=num2str(s16PropGainShift);
      |       if ~strcmp(s16PropGainShift_bkup,tmps)
      |         set_param(gcb,'s16PropGainShift',tmps);
      |       end
      |     end
      |     if isnan(s16IntegGainShift)
      |       if ~strcmp(s16IntegGainShift_bkup,'0')
      |         set_param(gcb,'s16IntegGainShift','0');
      |       end
      |     else
      |       tmps=num2str(s16IntegGainShift);
      |       if ~strcmp(s16IntegGainShift_bkup,tmps)
      |         set_param(gcb,'s16IntegGainShift',tmps);
      |       end
      |     end
      |     if isnan(s16DerivGainShift)
      |       if ~strcmp(s16DerivGainShift_bkup,'0')
      |         set_param(gcb,'s16DerivGainShift','0');
      |       end
      |     else
      |       tmps=num2str(s16DerivGainShift);
      |       if ~strcmp(s16DerivGainShift_bkup,tmps)
      |         set_param(gcb,'s16DerivGainShift',tmps);
      |       end
      |     end
      |     if isnan(f32LowerLimit)
      |       if ~strcmp(f32LowerLimit_bkup,'0')
      |         set_param(gcb,'f32LowerLimit','0');
      |       end
      |     else
      |       tmps=num2str(f32LowerLimit);
      |       if ~strcmp(f32LowerLimit_bkup,tmps)
      |         set_param(gcb,'f32LowerLimit',tmps);
      |       end
      |     end
      |     if isnan(f32UpperLimit)
      |       if ~strcmp(f32UpperLimit_bkup,'0')
      |         set_param(gcb,'f32UpperLimit','0');
      |       end
      |     else
      |       tmps=num2str(f32UpperLimit);
      |       if ~strcmp(f32UpperLimit_bkup,tmps)
      |         set_param(gcb,'f32UpperLimit',tmps);
      |       end
      |     end
      |   end
      | end
      mask Callback pgain:
      | autoCalcEn=get_param(gcb,'autoCalcEn');
      | if strcmp(autoCalcEn,'on')
      |   SampleTime=Simulink.data.evalinGlobal(bdroot,get_param(gcb,'SampleTime'));
      |   if (SampleTime==-1)
      |     SampleTime=str2double(get_param(gcb,'SampleTime_1'));
      |   end
      |   f32PropGain_bkup=get_param(gcb,'f32PropGain');
      |   f32IntegGain_bkup=get_param(gcb,'f32IntegGain');
      |   f32DerivGain_bkup=get_param(gcb,'f32DerivGain');
      |   f32FiltCoef_bkup=get_param(gcb,'f32FiltCoef');
      |   s16PropGainShift_bkup=get_param(gcb,'s16PropGainShift');
      |   s16IntegGainShift_bkup=get_param(gcb,'s16IntegGainShift');
      |   s16DerivGainShift_bkup=get_param(gcb,'s16DerivGainShift');
      |   f32LowerLimit_bkup=get_param(gcb,'f32LowerLimit');
      |   f32UpperLimit_bkup=get_param(gcb,'f32UpperLimit');
      |   pgain=Simulink.data.evalinGlobal(bdroot,get_param(gcb,'pgain'));
      |   igain=Simulink.data.evalinGlobal(bdroot,get_param(gcb,'igain'));
      |   dgain=Simulink.data.evalinGlobal(bdroot,get_param(gcb,'dgain'));
      |   filtCoef=Simulink.data.evalinGlobal(bdroot,get_param(gcb,'filtCoef'));
      |   lowerLimit=Simulink.data.evalinGlobal(bdroot,get_param(gcb,'lowerLimit'));
      |   upperLimit=Simulink.data.evalinGlobal(bdroot,get_param(gcb,'upperLimit'));
      |   inscale=Simulink.data.evalinGlobal(bdroot,get_param(gcb,'inscale'));
      |   outscale=Simulink.data.evalinGlobal(bdroot,get_param(gcb,'outscale'));
      |   if (upperLimit<=lowerLimit)
      |     warning('UpperLimit should be greater than LowerLimit.');
      |   end
      |   if (inscale<=0)
      |     warning('E_max must be positive.');
      |   end
      |   if (outscale<=0)
      |     warning('U_max must be positive.');
      |   end
      |   kpf=pgain*inscale/outscale;
      |   s16PropGainShift=ceil(log2(abs(kpf)));
      |   if s16PropGainShift<-31
      |     s16PropGainShift=-31;
      |   end
      |   if s16PropGainShift>31
      |     s16PropGainShift=31;
      |     warning(['Parameter s16PropGainShift of ' gcb ' exceeds the fixed-point range.']);
      |   end
      |   f32PropGain=round(kpf*2^(-s16PropGainShift)*2^31);
      |   if f32PropGain>2^31-1
      |     f32PropGain=2^31-1;
      |     warning(['Parameter f32PropGain of ' gcb ' exceeds the fixed-point range.']);
      |   end
      |   if f32PropGain<-2^31
      |     f32PropGain=-2^31;
      |     warning(['Parameter f32PropGain of ' gcb ' exceeds the fixed-point range.']);
      |   end
      |   kif=igain*SampleTime*0.5*inscale/outscale;
      |   s16IntegGainShift=ceil(log2(abs(kif)));
      |   if s16IntegGainShift<-31
      |     s16IntegGainShift=-31;
      |   end
      |   if s16IntegGainShift>31
      |     s16IntegGainShift=31;
      |     warning(['Parameter s16IntegGainShift of ' gcb ' exceeds the fixed-point range.']);
      |   end
      |   f32IntegGain=round(kif*2^(-s16IntegGainShift)*2^31);
      |   if f32IntegGain>2^31-1
      |     f32IntegGain=2^31-1;
      |     warning(['Parameter f32IntegGain of ' gcb ' exceeds the fixed-point range.']);
      |   end
      |   if f32IntegGain<-2^31
      |     f32IntegGain=-2^31;
      |     warning(['Parameter f32IntegGain of ' gcb ' exceeds the fixed-point range.']);
      |   end
      |   upperLimitf=upperLimit/outscale;
      |   lowerLimitf=lowerLimit/outscale;
      |   f32UpperLimit=round(upperLimitf*2^31);
      |   if f32UpperLimit>2^31-1
      |     f32UpperLimit=2^31-1;
      |     warning(['Parameter f32UpperLimit of ' gcb ' exceeds the fixed-point range.']);
      |   end
      |   if f32UpperLimit<-2^31
      |     f32UpperLimit=-2^31;
      |     warning(['Parameter f32UpperLimit of ' gcb ' exceeds the fixed-point range.']);
      |   end
      |   f32LowerLimit=round(lowerLimitf*2^31);
      |   if f32LowerLimit>2^31-1
      |     f32LowerLimit=2^31-1;
      |     warning(['Parameter f32LowerLimit of ' gcb ' exceeds the fixed-point range.']);
      |   end
      |   if f32LowerLimit<-2^31
      |     f32LowerLimit=-2^31;
      |     warning(['Parameter f32LowerLimit of ' gcb ' exceeds the fixed-point range.']);
      |   end
      |   exparg=-SampleTime*filtCoef;
      |   expconst=exp(exparg);
      |   f32FiltCoef=round(expconst*2^31);
      |   if f32FiltCoef>2^31-1
      |     f32FiltCoef=2^31-1;
      |     warning(['Parameter f32FiltCoef of ' gcb ' exceeds the fixed-point range.']);
      |   end
      |   if f32FiltCoef<-2^31
      |     f32FiltCoef=-2^31;
      |     warning(['Parameter f32FiltCoef of ' gcb ' exceeds the fixed-point range.']);
      |   end
      |   kdf=dgain/SampleTime*(1 - expconst)*inscale/outscale;
      |   s16DerivGainShift=ceil(log2(abs(kpf)));
      |   if s16DerivGainShift<-31
      |     s16DerivGainShift=-31;
      |   end
      |   if s16DerivGainShift>31
      |     s16DerivGainShift=31;
      |     warning(['Parameter s16DerivGainShift of ' gcb ' exceeds the fixed-point range.']);
      |   end
      |   f32DerivGain=round(kpf*2^(-s16DerivGainShift)*2^31);
      |   if f32DerivGain>2^31-1
      |     f32DerivGain=2^31-1;
      |     warning(['Parameter f32DerivGain of ' gcb ' exceeds the fixed-point range.']);
      |   end
      |   if f32DerivGain<-2^31
      |     f32DerivGain=-2^31;
      |     warning(['Parameter f32DerivGain of ' gcb ' exceeds the fixed-point range.']);
      |   end
      |   if isnan(f32PropGain)
      |     if ~strcmp(f32PropGain_bkup,'0')
      |       set_param(gcb,'f32PropGain','0');
      |     end
      |   else
      |     tmps=num2str(f32PropGain);
      |     if ~strcmp(f32PropGain_bkup,tmps)
      |       set_param(gcb,'f32PropGain',tmps);
      |     end
      |   end
      |   if isnan(f32IntegGain)
      |     if ~strcmp(f32IntegGain_bkup,'0')
      |       set_param(gcb,'f32IntegGain','0');
      |     end
      |   else
      |     tmps=num2str(f32IntegGain);
      |     if ~strcmp(f32IntegGain_bkup,tmps)
      |       set_param(gcb,'f32IntegGain',tmps);
      |     end
      |   end
      |   if isnan(f32DerivGain)
      |     if ~strcmp(f32DerivGain_bkup,'0')
      |       set_param(gcb,'f32DerivGain','0');
      |     end
      |   else
      |     tmps=num2str(f32DerivGain);
      |     if ~strcmp(f32DerivGain_bkup,tmps)
      |       set_param(gcb,'f32DerivGain',tmps);
      |     end
      |   end
      |   if isnan(f32FiltCoef)
      |     if ~strcmp(f32FiltCoef_bkup,'0')
      |       set_param(gcb,'f32FiltCoef','0');
      |     end
      |   else
      |     tmps=num2str(f32FiltCoef);
      |     if ~strcmp(f32FiltCoef_bkup,tmps)
      |       set_param(gcb,'f32FiltCoef',tmps);
      |     end
      |   end
      |   if isnan(s16PropGainShift)
      |     if ~strcmp(s16PropGainShift_bkup,'0')
      |       set_param(gcb,'s16PropGainShift','0');
      |     end
      |   else
      |     tmps=num2str(s16PropGainShift);
      |     if ~strcmp(s16PropGainShift_bkup,tmps)
      |       set_param(gcb,'s16PropGainShift',tmps);
      |     end
      |   end
      |   if isnan(s16IntegGainShift)
      |     if ~strcmp(s16IntegGainShift_bkup,'0')
      |       set_param(gcb,'s16IntegGainShift','0');
      |     end
      |   else
      |     tmps=num2str(s16IntegGainShift);
      |     if ~strcmp(s16IntegGainShift_bkup,tmps)
      |       set_param(gcb,'s16IntegGainShift',tmps);
      |     end
      |   end
      |   if isnan(s16DerivGainShift)
      |     if ~strcmp(s16DerivGainShift_bkup,'0')
      |       set_param(gcb,'s16DerivGainShift','0');
      |     end
      |   else
      |     tmps=num2str(s16DerivGainShift);
      |     if ~strcmp(s16DerivGainShift_bkup,tmps)
      |       set_param(gcb,'s16DerivGainShift',tmps);
      |     end
      |   end
      |   if isnan(f32LowerLimit)
      |     if ~strcmp(f32LowerLimit_bkup,'0')
      |       set_param(gcb,'f32LowerLimit','0');
      |     end
      |   else
      |     tmps=num2str(f32LowerLimit);
      |     if ~strcmp(f32LowerLimit_bkup,tmps)
      |       set_param(gcb,'f32LowerLimit',tmps);
      |     end
      |   end
      |   if isnan(f32UpperLimit)
      |     if ~strcmp(f32UpperLimit_bkup,'0')
      |       set_param(gcb,'f32UpperLimit','0');
      |     end
      |   else
      |     tmps=num2str(f32UpperLimit);
      |     if ~strcmp(f32UpperLimit_bkup,tmps)
      |       set_param(gcb,'f32UpperLimit',tmps);
      |     end
      |   end
      | end
      mask Callback igain:
      | autoCalcEn=get_param(gcb,'autoCalcEn');
      | if strcmp(autoCalcEn,'on')
      |   SampleTime=Simulink.data.evalinGlobal(bdroot,get_param(gcb,'SampleTime'));
      |   if (SampleTime==-1)
      |     SampleTime=str2double(get_param(gcb,'SampleTime_1'));
      |   end
      |   f32PropGain_bkup=get_param(gcb,'f32PropGain');
      |   f32IntegGain_bkup=get_param(gcb,'f32IntegGain');
      |   f32DerivGain_bkup=get_param(gcb,'f32DerivGain');
      |   f32FiltCoef_bkup=get_param(gcb,'f32FiltCoef');
      |   s16PropGainShift_bkup=get_param(gcb,'s16PropGainShift');
      |   s16IntegGainShift_bkup=get_param(gcb,'s16IntegGainShift');
      |   s16DerivGainShift_bkup=get_param(gcb,'s16DerivGainShift');
      |   f32LowerLimit_bkup=get_param(gcb,'f32LowerLimit');
      |   f32UpperLimit_bkup=get_param(gcb,'f32UpperLimit');
      |   pgain=Simulink.data.evalinGlobal(bdroot,get_param(gcb,'pgain'));
      |   igain=Simulink.data.evalinGlobal(bdroot,get_param(gcb,'igain'));
      |   dgain=Simulink.data.evalinGlobal(bdroot,get_param(gcb,'dgain'));
      |   filtCoef=Simulink.data.evalinGlobal(bdroot,get_param(gcb,'filtCoef'));
      |   lowerLimit=Simulink.data.evalinGlobal(bdroot,get_param(gcb,'lowerLimit'));
      |   upperLimit=Simulink.data.evalinGlobal(bdroot,get_param(gcb,'upperLimit'));
      |   inscale=Simulink.data.evalinGlobal(bdroot,get_param(gcb,'inscale'));
      |   outscale=Simulink.data.evalinGlobal(bdroot,get_param(gcb,'outscale'));
      |   if (upperLimit<=lowerLimit)
      |     warning('UpperLimit should be greater than LowerLimit.');
      |   end
      |   if (inscale<=0)
      |     warning('E_max must be positive.');
      |   end
      |   if (outscale<=0)
      |     warning('U_max must be positive.');
      |   end
      |   kpf=pgain*inscale/outscale;
      |   s16PropGainShift=ceil(log2(abs(kpf)));
      |   if s16PropGainShift<-31
      |     s16PropGainShift=-31;
      |   end
      |   if s16PropGainShift>31
      |     s16PropGainShift=31;
      |     warning(['Parameter s16PropGainShift of ' gcb ' exceeds the fixed-point range.']);
      |   end
      |   f32PropGain=round(kpf*2^(-s16PropGainShift)*2^31);
      |   if f32PropGain>2^31-1
      |     f32PropGain=2^31-1;
      |     warning(['Parameter f32PropGain of ' gcb ' exceeds the fixed-point range.']);
      |   end
      |   if f32PropGain<-2^31
      |     f32PropGain=-2^31;
      |     warning(['Parameter f32PropGain of ' gcb ' exceeds the fixed-point range.']);
      |   end
      |   kif=igain*SampleTime*0.5*inscale/outscale;
      |   s16IntegGainShift=ceil(log2(abs(kif)));
      |   if s16IntegGainShift<-31
      |     s16IntegGainShift=-31;
      |   end
      |   if s16IntegGainShift>31
      |     s16IntegGainShift=31;
      |     warning(['Parameter s16IntegGainShift of ' gcb ' exceeds the fixed-point range.']);
      |   end
      |   f32IntegGain=round(kif*2^(-s16IntegGainShift)*2^31);
      |   if f32IntegGain>2^31-1
      |     f32IntegGain=2^31-1;
      |     warning(['Parameter f32IntegGain of ' gcb ' exceeds the fixed-point range.']);
      |   end
      |   if f32IntegGain<-2^31
      |     f32IntegGain=-2^31;
      |     warning(['Parameter f32IntegGain of ' gcb ' exceeds the fixed-point range.']);
      |   end
      |   upperLimitf=upperLimit/outscale;
      |   lowerLimitf=lowerLimit/outscale;
      |   f32UpperLimit=round(upperLimitf*2^31);
      |   if f32UpperLimit>2^31-1
      |     f32UpperLimit=2^31-1;
      |     warning(['Parameter f32UpperLimit of ' gcb ' exceeds the fixed-point range.']);
      |   end
      |   if f32UpperLimit<-2^31
      |     f32UpperLimit=-2^31;
      |     warning(['Parameter f32UpperLimit of ' gcb ' exceeds the fixed-point range.']);
      |   end
      |   f32LowerLimit=round(lowerLimitf*2^31);
      |   if f32LowerLimit>2^31-1
      |     f32LowerLimit=2^31-1;
      |     warning(['Parameter f32LowerLimit of ' gcb ' exceeds the fixed-point range.']);
      |   end
      |   if f32LowerLimit<-2^31
      |     f32LowerLimit=-2^31;
      |     warning(['Parameter f32LowerLimit of ' gcb ' exceeds the fixed-point range.']);
      |   end
      |   exparg=-SampleTime*filtCoef;
      |   expconst=exp(exparg);
      |   f32FiltCoef=round(expconst*2^31);
      |   if f32FiltCoef>2^31-1
      |     f32FiltCoef=2^31-1;
      |     warning(['Parameter f32FiltCoef of ' gcb ' exceeds the fixed-point range.']);
      |   end
      |   if f32FiltCoef<-2^31
      |     f32FiltCoef=-2^31;
      |     warning(['Parameter f32FiltCoef of ' gcb ' exceeds the fixed-point range.']);
      |   end
      |   kdf=dgain/SampleTime*(1 - expconst)*inscale/outscale;
      |   s16DerivGainShift=ceil(log2(abs(kpf)));
      |   if s16DerivGainShift<-31
      |     s16DerivGainShift=-31;
      |   end
      |   if s16DerivGainShift>31
      |     s16DerivGainShift=31;
      |     warning(['Parameter s16DerivGainShift of ' gcb ' exceeds the fixed-point range.']);
      |   end
      |   f32DerivGain=round(kpf*2^(-s16DerivGainShift)*2^31);
      |   if f32DerivGain>2^31-1
      |     f32DerivGain=2^31-1;
      |     warning(['Parameter f32DerivGain of ' gcb ' exceeds the fixed-point range.']);
      |   end
      |   if f32DerivGain<-2^31
      |     f32DerivGain=-2^31;
      |     warning(['Parameter f32DerivGain of ' gcb ' exceeds the fixed-point range.']);
      |   end
      |   if isnan(f32PropGain)
      |     if ~strcmp(f32PropGain_bkup,'0')
      |       set_param(gcb,'f32PropGain','0');
      |     end
      |   else
      |     tmps=num2str(f32PropGain);
      |     if ~strcmp(f32PropGain_bkup,tmps)
      |       set_param(gcb,'f32PropGain',tmps);
      |     end
      |   end
      |   if isnan(f32IntegGain)
      |     if ~strcmp(f32IntegGain_bkup,'0')
      |       set_param(gcb,'f32IntegGain','0');
      |     end
      |   else
      |     tmps=num2str(f32IntegGain);
      |     if ~strcmp(f32IntegGain_bkup,tmps)
      |       set_param(gcb,'f32IntegGain',tmps);
      |     end
      |   end
      |   if isnan(f32DerivGain)
      |     if ~strcmp(f32DerivGain_bkup,'0')
      |       set_param(gcb,'f32DerivGain','0');
      |     end
      |   else
      |     tmps=num2str(f32DerivGain);
      |     if ~strcmp(f32DerivGain_bkup,tmps)
      |       set_param(gcb,'f32DerivGain',tmps);
      |     end
      |   end
      |   if isnan(f32FiltCoef)
      |     if ~strcmp(f32FiltCoef_bkup,'0')
      |       set_param(gcb,'f32FiltCoef','0');
      |     end
      |   else
      |     tmps=num2str(f32FiltCoef);
      |     if ~strcmp(f32FiltCoef_bkup,tmps)
      |       set_param(gcb,'f32FiltCoef',tmps);
      |     end
      |   end
      |   if isnan(s16PropGainShift)
      |     if ~strcmp(s16PropGainShift_bkup,'0')
      |       set_param(gcb,'s16PropGainShift','0');
      |     end
      |   else
      |     tmps=num2str(s16PropGainShift);
      |     if ~strcmp(s16PropGainShift_bkup,tmps)
      |       set_param(gcb,'s16PropGainShift',tmps);
      |     end
      |   end
      |   if isnan(s16IntegGainShift)
      |     if ~strcmp(s16IntegGainShift_bkup,'0')
      |       set_param(gcb,'s16IntegGainShift','0');
      |     end
      |   else
      |     tmps=num2str(s16IntegGainShift);
      |     if ~strcmp(s16IntegGainShift_bkup,tmps)
      |       set_param(gcb,'s16IntegGainShift',tmps);
      |     end
      |   end
      |   if isnan(s16DerivGainShift)
      |     if ~strcmp(s16DerivGainShift_bkup,'0')
      |       set_param(gcb,'s16DerivGainShift','0');
      |     end
      |   else
      |     tmps=num2str(s16DerivGainShift);
      |     if ~strcmp(s16DerivGainShift_bkup,tmps)
      |       set_param(gcb,'s16DerivGainShift',tmps);
      |     end
      |   end
      |   if isnan(f32LowerLimit)
      |     if ~strcmp(f32LowerLimit_bkup,'0')
      |       set_param(gcb,'f32LowerLimit','0');
      |     end
      |   else
      |     tmps=num2str(f32LowerLimit);
      |     if ~strcmp(f32LowerLimit_bkup,tmps)
      |       set_param(gcb,'f32LowerLimit',tmps);
      |     end
      |   end
      |   if isnan(f32UpperLimit)
      |     if ~strcmp(f32UpperLimit_bkup,'0')
      |       set_param(gcb,'f32UpperLimit','0');
      |     end
      |   else
      |     tmps=num2str(f32UpperLimit);
      |     if ~strcmp(f32UpperLimit_bkup,tmps)
      |       set_param(gcb,'f32UpperLimit',tmps);
      |     end
      |   end
      | end
      mask Callback dgain:
      | autoCalcEn=get_param(gcb,'autoCalcEn');
      | if strcmp(autoCalcEn,'on')
      |   SampleTime=Simulink.data.evalinGlobal(bdroot,get_param(gcb,'SampleTime'));
      |   if (SampleTime==-1)
      |     SampleTime=str2double(get_param(gcb,'SampleTime_1'));
      |   end
      |   f32PropGain_bkup=get_param(gcb,'f32PropGain');
      |   f32IntegGain_bkup=get_param(gcb,'f32IntegGain');
      |   f32DerivGain_bkup=get_param(gcb,'f32DerivGain');
      |   f32FiltCoef_bkup=get_param(gcb,'f32FiltCoef');
      |   s16PropGainShift_bkup=get_param(gcb,'s16PropGainShift');
      |   s16IntegGainShift_bkup=get_param(gcb,'s16IntegGainShift');
      |   s16DerivGainShift_bkup=get_param(gcb,'s16DerivGainShift');
      |   f32LowerLimit_bkup=get_param(gcb,'f32LowerLimit');
      |   f32UpperLimit_bkup=get_param(gcb,'f32UpperLimit');
      |   pgain=Simulink.data.evalinGlobal(bdroot,get_param(gcb,'pgain'));
      |   igain=Simulink.data.evalinGlobal(bdroot,get_param(gcb,'igain'));
      |   dgain=Simulink.data.evalinGlobal(bdroot,get_param(gcb,'dgain'));
      |   filtCoef=Simulink.data.evalinGlobal(bdroot,get_param(gcb,'filtCoef'));
      |   lowerLimit=Simulink.data.evalinGlobal(bdroot,get_param(gcb,'lowerLimit'));
      |   upperLimit=Simulink.data.evalinGlobal(bdroot,get_param(gcb,'upperLimit'));
      |   inscale=Simulink.data.evalinGlobal(bdroot,get_param(gcb,'inscale'));
      |   outscale=Simulink.data.evalinGlobal(bdroot,get_param(gcb,'outscale'));
      |   if (upperLimit<=lowerLimit)
      |     warning('UpperLimit should be greater than LowerLimit.');
      |   end
      |   if (inscale<=0)
      |     warning('E_max must be positive.');
      |   end
      |   if (outscale<=0)
      |     warning('U_max must be positive.');
      |   end
      |   kpf=pgain*inscale/outscale;
      |   s16PropGainShift=ceil(log2(abs(kpf)));
      |   if s16PropGainShift<-31
      |     s16PropGainShift=-31;
      |   end
      |   if s16PropGainShift>31
      |     s16PropGainShift=31;
      |     warning(['Parameter s16PropGainShift of ' gcb ' exceeds the fixed-point range.']);
      |   end
      |   f32PropGain=round(kpf*2^(-s16PropGainShift)*2^31);
      |   if f32PropGain>2^31-1
      |     f32PropGain=2^31-1;
      |     warning(['Parameter f32PropGain of ' gcb ' exceeds the fixed-point range.']);
      |   end
      |   if f32PropGain<-2^31
      |     f32PropGain=-2^31;
      |     warning(['Parameter f32PropGain of ' gcb ' exceeds the fixed-point range.']);
      |   end
      |   kif=igain*SampleTime*0.5*inscale/outscale;
      |   s16IntegGainShift=ceil(log2(abs(kif)));
      |   if s16IntegGainShift<-31
      |     s16IntegGainShift=-31;
      |   end
      |   if s16IntegGainShift>31
      |     s16IntegGainShift=31;
      |     warning(['Parameter s16IntegGainShift of ' gcb ' exceeds the fixed-point range.']);
      |   end
      |   f32IntegGain=round(kif*2^(-s16IntegGainShift)*2^31);
      |   if f32IntegGain>2^31-1
      |     f32IntegGain=2^31-1;
      |     warning(['Parameter f32IntegGain of ' gcb ' exceeds the fixed-point range.']);
      |   end
      |   if f32IntegGain<-2^31
      |     f32IntegGain=-2^31;
      |     warning(['Parameter f32IntegGain of ' gcb ' exceeds the fixed-point range.']);
      |   end
      |   upperLimitf=upperLimit/outscale;
      |   lowerLimitf=lowerLimit/outscale;
      |   f32UpperLimit=round(upperLimitf*2^31);
      |   if f32UpperLimit>2^31-1
      |     f32UpperLimit=2^31-1;
      |     warning(['Parameter f32UpperLimit of ' gcb ' exceeds the fixed-point range.']);
      |   end
      |   if f32UpperLimit<-2^31
      |     f32UpperLimit=-2^31;
      |     warning(['Parameter f32UpperLimit of ' gcb ' exceeds the fixed-point range.']);
      |   end
      |   f32LowerLimit=round(lowerLimitf*2^31);
      |   if f32LowerLimit>2^31-1
      |     f32LowerLimit=2^31-1;
      |     warning(['Parameter f32LowerLimit of ' gcb ' exceeds the fixed-point range.']);
      |   end
      |   if f32LowerLimit<-2^31
      |     f32LowerLimit=-2^31;
      |     warning(['Parameter f32LowerLimit of ' gcb ' exceeds the fixed-point range.']);
      |   end
      |   exparg=-SampleTime*filtCoef;
      |   expconst=exp(exparg);
      |   f32FiltCoef=round(expconst*2^31);
      |   if f32FiltCoef>2^31-1
      |     f32FiltCoef=2^31-1;
      |     warning(['Parameter f32FiltCoef of ' gcb ' exceeds the fixed-point range.']);
      |   end
      |   if f32FiltCoef<-2^31
      |     f32FiltCoef=-2^31;
      |     warning(['Parameter f32FiltCoef of ' gcb ' exceeds the fixed-point range.']);
      |   end
      |   kdf=dgain/SampleTime*(1 - expconst)*inscale/outscale;
      |   s16DerivGainShift=ceil(log2(abs(kpf)));
      |   if s16DerivGainShift<-31
      |     s16DerivGainShift=-31;
      |   end
      |   if s16DerivGainShift>31
      |     s16DerivGainShift=31;
      |     warning(['Parameter s16DerivGainShift of ' gcb ' exceeds the fixed-point range.']);
      |   end
      |   f32DerivGain=round(kpf*2^(-s16DerivGainShift)*2^31);
      |   if f32DerivGain>2^31-1
      |     f32DerivGain=2^31-1;
      |     warning(['Parameter f32DerivGain of ' gcb ' exceeds the fixed-point range.']);
      |   end
      |   if f32DerivGain<-2^31
      |     f32DerivGain=-2^31;
      |     warning(['Parameter f32DerivGain of ' gcb ' exceeds the fixed-point range.']);
      |   end
      |   if isnan(f32PropGain)
      |     if ~strcmp(f32PropGain_bkup,'0')
      |       set_param(gcb,'f32PropGain','0');
      |     end
      |   else
      |     tmps=num2str(f32PropGain);
      |     if ~strcmp(f32PropGain_bkup,tmps)
      |       set_param(gcb,'f32PropGain',tmps);
      |     end
      |   end
      |   if isnan(f32IntegGain)
      |     if ~strcmp(f32IntegGain_bkup,'0')
      |       set_param(gcb,'f32IntegGain','0');
      |     end
      |   else
      |     tmps=num2str(f32IntegGain);
      |     if ~strcmp(f32IntegGain_bkup,tmps)
      |       set_param(gcb,'f32IntegGain',tmps);
      |     end
      |   end
      |   if isnan(f32DerivGain)
      |     if ~strcmp(f32DerivGain_bkup,'0')
      |       set_param(gcb,'f32DerivGain','0');
      |     end
      |   else
      |     tmps=num2str(f32DerivGain);
      |     if ~strcmp(f32DerivGain_bkup,tmps)
      |       set_param(gcb,'f32DerivGain',tmps);
      |     end
      |   end
      |   if isnan(f32FiltCoef)
      |     if ~strcmp(f32FiltCoef_bkup,'0')
      |       set_param(gcb,'f32FiltCoef','0');
      |     end
      |   else
      |     tmps=num2str(f32FiltCoef);
      |     if ~strcmp(f32FiltCoef_bkup,tmps)
      |       set_param(gcb,'f32FiltCoef',tmps);
      |     end
      |   end
      |   if isnan(s16PropGainShift)
      |     if ~strcmp(s16PropGainShift_bkup,'0')
      |       set_param(gcb,'s16PropGainShift','0');
      |     end
      |   else
      |     tmps=num2str(s16PropGainShift);
      |     if ~strcmp(s16PropGainShift_bkup,tmps)
      |       set_param(gcb,'s16PropGainShift',tmps);
      |     end
      |   end
      |   if isnan(s16IntegGainShift)
      |     if ~strcmp(s16IntegGainShift_bkup,'0')
      |       set_param(gcb,'s16IntegGainShift','0');
      |     end
      |   else
      |     tmps=num2str(s16IntegGainShift);
      |     if ~strcmp(s16IntegGainShift_bkup,tmps)
      |       set_param(gcb,'s16IntegGainShift',tmps);
      |     end
      |   end
      |   if isnan(s16DerivGainShift)
      |     if ~strcmp(s16DerivGainShift_bkup,'0')
      |       set_param(gcb,'s16DerivGainShift','0');
      |     end
      |   else
      |     tmps=num2str(s16DerivGainShift);
      |     if ~strcmp(s16DerivGainShift_bkup,tmps)
      |       set_param(gcb,'s16DerivGainShift',tmps);
      |     end
      |   end
      |   if isnan(f32LowerLimit)
      |     if ~strcmp(f32LowerLimit_bkup,'0')
      |       set_param(gcb,'f32LowerLimit','0');
      |     end
      |   else
      |     tmps=num2str(f32LowerLimit);
      |     if ~strcmp(f32LowerLimit_bkup,tmps)
      |       set_param(gcb,'f32LowerLimit',tmps);
      |     end
      |   end
      |   if isnan(f32UpperLimit)
      |     if ~strcmp(f32UpperLimit_bkup,'0')
      |       set_param(gcb,'f32UpperLimit','0');
      |     end
      |   else
      |     tmps=num2str(f32UpperLimit);
      |     if ~strcmp(f32UpperLimit_bkup,tmps)
      |       set_param(gcb,'f32UpperLimit',tmps);
      |     end
      |   end
      | end
      mask Callback filtCoef:
      | autoCalcEn=get_param(gcb,'autoCalcEn');
      | if strcmp(autoCalcEn,'on')
      |   SampleTime=Simulink.data.evalinGlobal(bdroot,get_param(gcb,'SampleTime'));
      |   if (SampleTime==-1)
      |     SampleTime=str2double(get_param(gcb,'SampleTime_1'));
      |   end
      |   f32PropGain_bkup=get_param(gcb,'f32PropGain');
      |   f32IntegGain_bkup=get_param(gcb,'f32IntegGain');
      |   f32DerivGain_bkup=get_param(gcb,'f32DerivGain');
      |   f32FiltCoef_bkup=get_param(gcb,'f32FiltCoef');
      |   s16PropGainShift_bkup=get_param(gcb,'s16PropGainShift');
      |   s16IntegGainShift_bkup=get_param(gcb,'s16IntegGainShift');
      |   s16DerivGainShift_bkup=get_param(gcb,'s16DerivGainShift');
      |   f32LowerLimit_bkup=get_param(gcb,'f32LowerLimit');
      |   f32UpperLimit_bkup=get_param(gcb,'f32UpperLimit');
      |   pgain=Simulink.data.evalinGlobal(bdroot,get_param(gcb,'pgain'));
      |   igain=Simulink.data.evalinGlobal(bdroot,get_param(gcb,'igain'));
      |   dgain=Simulink.data.evalinGlobal(bdroot,get_param(gcb,'dgain'));
      |   filtCoef=Simulink.data.evalinGlobal(bdroot,get_param(gcb,'filtCoef'));
      |   lowerLimit=Simulink.data.evalinGlobal(bdroot,get_param(gcb,'lowerLimit'));
      |   upperLimit=Simulink.data.evalinGlobal(bdroot,get_param(gcb,'upperLimit'));
      |   inscale=Simulink.data.evalinGlobal(bdroot,get_param(gcb,'inscale'));
      |   outscale=Simulink.data.evalinGlobal(bdroot,get_param(gcb,'outscale'));
      |   if (upperLimit<=lowerLimit)
      |     warning('UpperLimit should be greater than LowerLimit.');
      |   end
      |   if (inscale<=0)
      |     warning('E_max must be positive.');
      |   end
      |   if (outscale<=0)
      |     warning('U_max must be positive.');
      |   end
      |   kpf=pgain*inscale/outscale;
      |   s16PropGainShift=ceil(log2(abs(kpf)));
      |   if s16PropGainShift<-31
      |     s16PropGainShift=-31;
      |   end
      |   if s16PropGainShift>31
      |     s16PropGainShift=31;
      |     warning(['Parameter s16PropGainShift of ' gcb ' exceeds the fixed-point range.']);
      |   end
      |   f32PropGain=round(kpf*2^(-s16PropGainShift)*2^31);
      |   if f32PropGain>2^31-1
      |     f32PropGain=2^31-1;
      |     warning(['Parameter f32PropGain of ' gcb ' exceeds the fixed-point range.']);
      |   end
      |   if f32PropGain<-2^31
      |     f32PropGain=-2^31;
      |     warning(['Parameter f32PropGain of ' gcb ' exceeds the fixed-point range.']);
      |   end
      |   kif=igain*SampleTime*0.5*inscale/outscale;
      |   s16IntegGainShift=ceil(log2(abs(kif)));
      |   if s16IntegGainShift<-31
      |     s16IntegGainShift=-31;
      |   end
      |   if s16IntegGainShift>31
      |     s16IntegGainShift=31;
      |     warning(['Parameter s16IntegGainShift of ' gcb ' exceeds the fixed-point range.']);
      |   end
      |   f32IntegGain=round(kif*2^(-s16IntegGainShift)*2^31);
      |   if f32IntegGain>2^31-1
      |     f32IntegGain=2^31-1;
      |     warning(['Parameter f32IntegGain of ' gcb ' exceeds the fixed-point range.']);
      |   end
      |   if f32IntegGain<-2^31
      |     f32IntegGain=-2^31;
      |     warning(['Parameter f32IntegGain of ' gcb ' exceeds the fixed-point range.']);
      |   end
      |   upperLimitf=upperLimit/outscale;
      |   lowerLimitf=lowerLimit/outscale;
      |   f32UpperLimit=round(upperLimitf*2^31);
      |   if f32UpperLimit>2^31-1
      |     f32UpperLimit=2^31-1;
      |     warning(['Parameter f32UpperLimit of ' gcb ' exceeds the fixed-point range.']);
      |   end
      |   if f32UpperLimit<-2^31
      |     f32UpperLimit=-2^31;
      |     warning(['Parameter f32UpperLimit of ' gcb ' exceeds the fixed-point range.']);
      |   end
      |   f32LowerLimit=round(lowerLimitf*2^31);
      |   if f32LowerLimit>2^31-1
      |     f32LowerLimit=2^31-1;
      |     warning(['Parameter f32LowerLimit of ' gcb ' exceeds the fixed-point range.']);
      |   end
      |   if f32LowerLimit<-2^31
      |     f32LowerLimit=-2^31;
      |     warning(['Parameter f32LowerLimit of ' gcb ' exceeds the fixed-point range.']);
      |   end
      |   exparg=-SampleTime*filtCoef;
      |   expconst=exp(exparg);
      |   f32FiltCoef=round(expconst*2^31);
      |   if f32FiltCoef>2^31-1
      |     f32FiltCoef=2^31-1;
      |     warning(['Parameter f32FiltCoef of ' gcb ' exceeds the fixed-point range.']);
      |   end
      |   if f32FiltCoef<-2^31
      |     f32FiltCoef=-2^31;
      |     warning(['Parameter f32FiltCoef of ' gcb ' exceeds the fixed-point range.']);
      |   end
      |   kdf=dgain/SampleTime*(1 - expconst)*inscale/outscale;
      |   s16DerivGainShift=ceil(log2(abs(kpf)));
      |   if s16DerivGainShift<-31
      |     s16DerivGainShift=-31;
      |   end
      |   if s16DerivGainShift>31
      |     s16DerivGainShift=31;
      |     warning(['Parameter s16DerivGainShift of ' gcb ' exceeds the fixed-point range.']);
      |   end
      |   f32DerivGain=round(kpf*2^(-s16DerivGainShift)*2^31);
      |   if f32DerivGain>2^31-1
      |     f32DerivGain=2^31-1;
      |     warning(['Parameter f32DerivGain of ' gcb ' exceeds the fixed-point range.']);
      |   end
      |   if f32DerivGain<-2^31
      |     f32DerivGain=-2^31;
      |     warning(['Parameter f32DerivGain of ' gcb ' exceeds the fixed-point range.']);
      |   end
      |   if isnan(f32PropGain)
      |     if ~strcmp(f32PropGain_bkup,'0')
      |       set_param(gcb,'f32PropGain','0');
      |     end
      |   else
      |     tmps=num2str(f32PropGain);
      |     if ~strcmp(f32PropGain_bkup,tmps)
      |       set_param(gcb,'f32PropGain',tmps);
      |     end
      |   end
      |   if isnan(f32IntegGain)
      |     if ~strcmp(f32IntegGain_bkup,'0')
      |       set_param(gcb,'f32IntegGain','0');
      |     end
      |   else
      |     tmps=num2str(f32IntegGain);
      |     if ~strcmp(f32IntegGain_bkup,tmps)
      |       set_param(gcb,'f32IntegGain',tmps);
      |     end
      |   end
      |   if isnan(f32DerivGain)
      |     if ~strcmp(f32DerivGain_bkup,'0')
      |       set_param(gcb,'f32DerivGain','0');
      |     end
      |   else
      |     tmps=num2str(f32DerivGain);
      |     if ~strcmp(f32DerivGain_bkup,tmps)
      |       set_param(gcb,'f32DerivGain',tmps);
      |     end
      |   end
      |   if isnan(f32FiltCoef)
      |     if ~strcmp(f32FiltCoef_bkup,'0')
      |       set_param(gcb,'f32FiltCoef','0');
      |     end
      |   else
      |     tmps=num2str(f32FiltCoef);
      |     if ~strcmp(f32FiltCoef_bkup,tmps)
      |       set_param(gcb,'f32FiltCoef',tmps);
      |     end
      |   end
      |   if isnan(s16PropGainShift)
      |     if ~strcmp(s16PropGainShift_bkup,'0')
      |       set_param(gcb,'s16PropGainShift','0');
      |     end
      |   else
      |     tmps=num2str(s16PropGainShift);
      |     if ~strcmp(s16PropGainShift_bkup,tmps)
      |       set_param(gcb,'s16PropGainShift',tmps);
      |     end
      |   end
      |   if isnan(s16IntegGainShift)
      |     if ~strcmp(s16IntegGainShift_bkup,'0')
      |       set_param(gcb,'s16IntegGainShift','0');
      |     end
      |   else
      |     tmps=num2str(s16IntegGainShift);
      |     if ~strcmp(s16IntegGainShift_bkup,tmps)
      |       set_param(gcb,'s16IntegGainShift',tmps);
      |     end
      |   end
      |   if isnan(s16DerivGainShift)
      |     if ~strcmp(s16DerivGainShift_bkup,'0')
      |       set_param(gcb,'s16DerivGainShift','0');
      |     end
      |   else
      |     tmps=num2str(s16DerivGainShift);
      |     if ~strcmp(s16DerivGainShift_bkup,tmps)
      |       set_param(gcb,'s16DerivGainShift',tmps);
      |     end
      |   end
      |   if isnan(f32LowerLimit)
      |     if ~strcmp(f32LowerLimit_bkup,'0')
      |       set_param(gcb,'f32LowerLimit','0');
      |     end
      |   else
      |     tmps=num2str(f32LowerLimit);
      |     if ~strcmp(f32LowerLimit_bkup,tmps)
      |       set_param(gcb,'f32LowerLimit',tmps);
      |     end
      |   end
      |   if isnan(f32UpperLimit)
      |     if ~strcmp(f32UpperLimit_bkup,'0')
      |       set_param(gcb,'f32UpperLimit','0');
      |     end
      |   else
      |     tmps=num2str(f32UpperLimit);
      |     if ~strcmp(f32UpperLimit_bkup,tmps)
      |       set_param(gcb,'f32UpperLimit',tmps);
      |     end
      |   end
      | end
      mask Callback lowerLimit:
      | autoCalcEn=get_param(gcb,'autoCalcEn');
      | if strcmp(autoCalcEn,'on')
      |   SampleTime=Simulink.data.evalinGlobal(bdroot,get_param(gcb,'SampleTime'));
      |   if (SampleTime==-1)
      |     SampleTime=str2double(get_param(gcb,'SampleTime_1'));
      |   end
      |   f32PropGain_bkup=get_param(gcb,'f32PropGain');
      |   f32IntegGain_bkup=get_param(gcb,'f32IntegGain');
      |   f32DerivGain_bkup=get_param(gcb,'f32DerivGain');
      |   f32FiltCoef_bkup=get_param(gcb,'f32FiltCoef');
      |   s16PropGainShift_bkup=get_param(gcb,'s16PropGainShift');
      |   s16IntegGainShift_bkup=get_param(gcb,'s16IntegGainShift');
      |   s16DerivGainShift_bkup=get_param(gcb,'s16DerivGainShift');
      |   f32LowerLimit_bkup=get_param(gcb,'f32LowerLimit');
      |   f32UpperLimit_bkup=get_param(gcb,'f32UpperLimit');
      |   pgain=Simulink.data.evalinGlobal(bdroot,get_param(gcb,'pgain'));
      |   igain=Simulink.data.evalinGlobal(bdroot,get_param(gcb,'igain'));
      |   dgain=Simulink.data.evalinGlobal(bdroot,get_param(gcb,'dgain'));
      |   filtCoef=Simulink.data.evalinGlobal(bdroot,get_param(gcb,'filtCoef'));
      |   lowerLimit=Simulink.data.evalinGlobal(bdroot,get_param(gcb,'lowerLimit'));
      |   upperLimit=Simulink.data.evalinGlobal(bdroot,get_param(gcb,'upperLimit'));
      |   inscale=Simulink.data.evalinGlobal(bdroot,get_param(gcb,'inscale'));
      |   outscale=Simulink.data.evalinGlobal(bdroot,get_param(gcb,'outscale'));
      |   if (upperLimit<=lowerLimit)
      |     warning('UpperLimit should be greater than LowerLimit.');
      |   end
      |   if (inscale<=0)
      |     warning('E_max must be positive.');
      |   end
      |   if (outscale<=0)
      |     warning('U_max must be positive.');
      |   end
      |   kpf=pgain*inscale/outscale;
      |   s16PropGainShift=ceil(log2(abs(kpf)));
      |   if s16PropGainShift<-31
      |     s16PropGainShift=-31;
      |   end
      |   if s16PropGainShift>31
      |     s16PropGainShift=31;
      |     warning(['Parameter s16PropGainShift of ' gcb ' exceeds the fixed-point range.']);
      |   end
      |   f32PropGain=round(kpf*2^(-s16PropGainShift)*2^31);
      |   if f32PropGain>2^31-1
      |     f32PropGain=2^31-1;
      |     warning(['Parameter f32PropGain of ' gcb ' exceeds the fixed-point range.']);
      |   end
      |   if f32PropGain<-2^31
      |     f32PropGain=-2^31;
      |     warning(['Parameter f32PropGain of ' gcb ' exceeds the fixed-point range.']);
      |   end
      |   kif=igain*SampleTime*0.5*inscale/outscale;
      |   s16IntegGainShift=ceil(log2(abs(kif)));
      |   if s16IntegGainShift<-31
      |     s16IntegGainShift=-31;
      |   end
      |   if s16IntegGainShift>31
      |     s16IntegGainShift=31;
      |     warning(['Parameter s16IntegGainShift of ' gcb ' exceeds the fixed-point range.']);
      |   end
      |   f32IntegGain=round(kif*2^(-s16IntegGainShift)*2^31);
      |   if f32IntegGain>2^31-1
      |     f32IntegGain=2^31-1;
      |     warning(['Parameter f32IntegGain of ' gcb ' exceeds the fixed-point range.']);
      |   end
      |   if f32IntegGain<-2^31
      |     f32IntegGain=-2^31;
      |     warning(['Parameter f32IntegGain of ' gcb ' exceeds the fixed-point range.']);
      |   end
      |   upperLimitf=upperLimit/outscale;
      |   lowerLimitf=lowerLimit/outscale;
      |   f32UpperLimit=round(upperLimitf*2^31);
      |   if f32UpperLimit>2^31-1
      |     f32UpperLimit=2^31-1;
      |     warning(['Parameter f32UpperLimit of ' gcb ' exceeds the fixed-point range.']);
      |   end
      |   if f32UpperLimit<-2^31
      |     f32UpperLimit=-2^31;
      |     warning(['Parameter f32UpperLimit of ' gcb ' exceeds the fixed-point range.']);
      |   end
      |   f32LowerLimit=round(lowerLimitf*2^31);
      |   if f32LowerLimit>2^31-1
      |     f32LowerLimit=2^31-1;
      |     warning(['Parameter f32LowerLimit of ' gcb ' exceeds the fixed-point range.']);
      |   end
      |   if f32LowerLimit<-2^31
      |     f32LowerLimit=-2^31;
      |     warning(['Parameter f32LowerLimit of ' gcb ' exceeds the fixed-point range.']);
      |   end
      |   exparg=-SampleTime*filtCoef;
      |   expconst=exp(exparg);
      |   f32FiltCoef=round(expconst*2^31);
      |   if f32FiltCoef>2^31-1
      |     f32FiltCoef=2^31-1;
      |     warning(['Parameter f32FiltCoef of ' gcb ' exceeds the fixed-point range.']);
      |   end
      |   if f32FiltCoef<-2^31
      |     f32FiltCoef=-2^31;
      |     warning(['Parameter f32FiltCoef of ' gcb ' exceeds the fixed-point range.']);
      |   end
      |   kdf=dgain/SampleTime*(1 - expconst)*inscale/outscale;
      |   s16DerivGainShift=ceil(log2(abs(kpf)));
      |   if s16DerivGainShift<-31
      |     s16DerivGainShift=-31;
      |   end
      |   if s16DerivGainShift>31
      |     s16DerivGainShift=31;
      |     warning(['Parameter s16DerivGainShift of ' gcb ' exceeds the fixed-point range.']);
      |   end
      |   f32DerivGain=round(kpf*2^(-s16DerivGainShift)*2^31);
      |   if f32DerivGain>2^31-1
      |     f32DerivGain=2^31-1;
      |     warning(['Parameter f32DerivGain of ' gcb ' exceeds the fixed-point range.']);
      |   end
      |   if f32DerivGain<-2^31
      |     f32DerivGain=-2^31;
      |     warning(['Parameter f32DerivGain of ' gcb ' exceeds the fixed-point range.']);
      |   end
      |   if isnan(f32PropGain)
      |     if ~strcmp(f32PropGain_bkup,'0')
      |       set_param(gcb,'f32PropGain','0');
      |     end
      |   else
      |     tmps=num2str(f32PropGain);
      |     if ~strcmp(f32PropGain_bkup,tmps)
      |       set_param(gcb,'f32PropGain',tmps);
      |     end
      |   end
      |   if isnan(f32IntegGain)
      |     if ~strcmp(f32IntegGain_bkup,'0')
      |       set_param(gcb,'f32IntegGain','0');
      |     end
      |   else
      |     tmps=num2str(f32IntegGain);
      |     if ~strcmp(f32IntegGain_bkup,tmps)
      |       set_param(gcb,'f32IntegGain',tmps);
      |     end
      |   end
      |   if isnan(f32DerivGain)
      |     if ~strcmp(f32DerivGain_bkup,'0')
      |       set_param(gcb,'f32DerivGain','0');
      |     end
      |   else
      |     tmps=num2str(f32DerivGain);
      |     if ~strcmp(f32DerivGain_bkup,tmps)
      |       set_param(gcb,'f32DerivGain',tmps);
      |     end
      |   end
      |   if isnan(f32FiltCoef)
      |     if ~strcmp(f32FiltCoef_bkup,'0')
      |       set_param(gcb,'f32FiltCoef','0');
      |     end
      |   else
      |     tmps=num2str(f32FiltCoef);
      |     if ~strcmp(f32FiltCoef_bkup,tmps)
      |       set_param(gcb,'f32FiltCoef',tmps);
      |     end
      |   end
      |   if isnan(s16PropGainShift)
      |     if ~strcmp(s16PropGainShift_bkup,'0')
      |       set_param(gcb,'s16PropGainShift','0');
      |     end
      |   else
      |     tmps=num2str(s16PropGainShift);
      |     if ~strcmp(s16PropGainShift_bkup,tmps)
      |       set_param(gcb,'s16PropGainShift',tmps);
      |     end
      |   end
      |   if isnan(s16IntegGainShift)
      |     if ~strcmp(s16IntegGainShift_bkup,'0')
      |       set_param(gcb,'s16IntegGainShift','0');
      |     end
      |   else
      |     tmps=num2str(s16IntegGainShift);
      |     if ~strcmp(s16IntegGainShift_bkup,tmps)
      |       set_param(gcb,'s16IntegGainShift',tmps);
      |     end
      |   end
      |   if isnan(s16DerivGainShift)
      |     if ~strcmp(s16DerivGainShift_bkup,'0')
      |       set_param(gcb,'s16DerivGainShift','0');
      |     end
      |   else
      |     tmps=num2str(s16DerivGainShift);
      |     if ~strcmp(s16DerivGainShift_bkup,tmps)
      |       set_param(gcb,'s16DerivGainShift',tmps);
      |     end
      |   end
      |   if isnan(f32LowerLimit)
      |     if ~strcmp(f32LowerLimit_bkup,'0')
      |       set_param(gcb,'f32LowerLimit','0');
      |     end
      |   else
      |     tmps=num2str(f32LowerLimit);
      |     if ~strcmp(f32LowerLimit_bkup,tmps)
      |       set_param(gcb,'f32LowerLimit',tmps);
      |     end
      |   end
      |   if isnan(f32UpperLimit)
      |     if ~strcmp(f32UpperLimit_bkup,'0')
      |       set_param(gcb,'f32UpperLimit','0');
      |     end
      |   else
      |     tmps=num2str(f32UpperLimit);
      |     if ~strcmp(f32UpperLimit_bkup,tmps)
      |       set_param(gcb,'f32UpperLimit',tmps);
      |     end
      |   end
      | end
      mask Callback upperLimit:
      | autoCalcEn=get_param(gcb,'autoCalcEn');
      | if strcmp(autoCalcEn,'on')
      |   SampleTime=Simulink.data.evalinGlobal(bdroot,get_param(gcb,'SampleTime'));
      |   if (SampleTime==-1)
      |     SampleTime=str2double(get_param(gcb,'SampleTime_1'));
      |   end
      |   f32PropGain_bkup=get_param(gcb,'f32PropGain');
      |   f32IntegGain_bkup=get_param(gcb,'f32IntegGain');
      |   f32DerivGain_bkup=get_param(gcb,'f32DerivGain');
      |   f32FiltCoef_bkup=get_param(gcb,'f32FiltCoef');
      |   s16PropGainShift_bkup=get_param(gcb,'s16PropGainShift');
      |   s16IntegGainShift_bkup=get_param(gcb,'s16IntegGainShift');
      |   s16DerivGainShift_bkup=get_param(gcb,'s16DerivGainShift');
      |   f32LowerLimit_bkup=get_param(gcb,'f32LowerLimit');
      |   f32UpperLimit_bkup=get_param(gcb,'f32UpperLimit');
      |   pgain=Simulink.data.evalinGlobal(bdroot,get_param(gcb,'pgain'));
      |   igain=Simulink.data.evalinGlobal(bdroot,get_param(gcb,'igain'));
      |   dgain=Simulink.data.evalinGlobal(bdroot,get_param(gcb,'dgain'));
      |   filtCoef=Simulink.data.evalinGlobal(bdroot,get_param(gcb,'filtCoef'));
      |   lowerLimit=Simulink.data.evalinGlobal(bdroot,get_param(gcb,'lowerLimit'));
      |   upperLimit=Simulink.data.evalinGlobal(bdroot,get_param(gcb,'upperLimit'));
      |   inscale=Simulink.data.evalinGlobal(bdroot,get_param(gcb,'inscale'));
      |   outscale=Simulink.data.evalinGlobal(bdroot,get_param(gcb,'outscale'));
      |   if (upperLimit<=lowerLimit)
      |     warning('UpperLimit should be greater than LowerLimit.');
      |   end
      |   if (inscale<=0)
      |     warning('E_max must be positive.');
      |   end
      |   if (outscale<=0)
      |     warning('U_max must be positive.');
      |   end
      |   kpf=pgain*inscale/outscale;
      |   s16PropGainShift=ceil(log2(abs(kpf)));
      |   if s16PropGainShift<-31
      |     s16PropGainShift=-31;
      |   end
      |   if s16PropGainShift>31
      |     s16PropGainShift=31;
      |     warning(['Parameter s16PropGainShift of ' gcb ' exceeds the fixed-point range.']);
      |   end
      |   f32PropGain=round(kpf*2^(-s16PropGainShift)*2^31);
      |   if f32PropGain>2^31-1
      |     f32PropGain=2^31-1;
      |     warning(['Parameter f32PropGain of ' gcb ' exceeds the fixed-point range.']);
      |   end
      |   if f32PropGain<-2^31
      |     f32PropGain=-2^31;
      |     warning(['Parameter f32PropGain of ' gcb ' exceeds the fixed-point range.']);
      |   end
      |   kif=igain*SampleTime*0.5*inscale/outscale;
      |   s16IntegGainShift=ceil(log2(abs(kif)));
      |   if s16IntegGainShift<-31
      |     s16IntegGainShift=-31;
      |   end
      |   if s16IntegGainShift>31
      |     s16IntegGainShift=31;
      |     warning(['Parameter s16IntegGainShift of ' gcb ' exceeds the fixed-point range.']);
      |   end
      |   f32IntegGain=round(kif*2^(-s16IntegGainShift)*2^31);
      |   if f32IntegGain>2^31-1
      |     f32IntegGain=2^31-1;
      |     warning(['Parameter f32IntegGain of ' gcb ' exceeds the fixed-point range.']);
      |   end
      |   if f32IntegGain<-2^31
      |     f32IntegGain=-2^31;
      |     warning(['Parameter f32IntegGain of ' gcb ' exceeds the fixed-point range.']);
      |   end
      |   upperLimitf=upperLimit/outscale;
      |   lowerLimitf=lowerLimit/outscale;
      |   f32UpperLimit=round(upperLimitf*2^31);
      |   if f32UpperLimit>2^31-1
      |     f32UpperLimit=2^31-1;
      |     warning(['Parameter f32UpperLimit of ' gcb ' exceeds the fixed-point range.']);
      |   end
      |   if f32UpperLimit<-2^31
      |     f32UpperLimit=-2^31;
      |     warning(['Parameter f32UpperLimit of ' gcb ' exceeds the fixed-point range.']);
      |   end
      |   f32LowerLimit=round(lowerLimitf*2^31);
      |   if f32LowerLimit>2^31-1
      |     f32LowerLimit=2^31-1;
      |     warning(['Parameter f32LowerLimit of ' gcb ' exceeds the fixed-point range.']);
      |   end
      |   if f32LowerLimit<-2^31
      |     f32LowerLimit=-2^31;
      |     warning(['Parameter f32LowerLimit of ' gcb ' exceeds the fixed-point range.']);
      |   end
      |   exparg=-SampleTime*filtCoef;
      |   expconst=exp(exparg);
      |   f32FiltCoef=round(expconst*2^31);
      |   if f32FiltCoef>2^31-1
      |     f32FiltCoef=2^31-1;
      |     warning(['Parameter f32FiltCoef of ' gcb ' exceeds the fixed-point range.']);
      |   end
      |   if f32FiltCoef<-2^31
      |     f32FiltCoef=-2^31;
      |     warning(['Parameter f32FiltCoef of ' gcb ' exceeds the fixed-point range.']);
      |   end
      |   kdf=dgain/SampleTime*(1 - expconst)*inscale/outscale;
      |   s16DerivGainShift=ceil(log2(abs(kpf)));
      |   if s16DerivGainShift<-31
      |     s16DerivGainShift=-31;
      |   end
      |   if s16DerivGainShift>31
      |     s16DerivGainShift=31;
      |     warning(['Parameter s16DerivGainShift of ' gcb ' exceeds the fixed-point range.']);
      |   end
      |   f32DerivGain=round(kpf*2^(-s16DerivGainShift)*2^31);
      |   if f32DerivGain>2^31-1
      |     f32DerivGain=2^31-1;
      |     warning(['Parameter f32DerivGain of ' gcb ' exceeds the fixed-point range.']);
      |   end
      |   if f32DerivGain<-2^31
      |     f32DerivGain=-2^31;
      |     warning(['Parameter f32DerivGain of ' gcb ' exceeds the fixed-point range.']);
      |   end
      |   if isnan(f32PropGain)
      |     if ~strcmp(f32PropGain_bkup,'0')
      |       set_param(gcb,'f32PropGain','0');
      |     end
      |   else
      |     tmps=num2str(f32PropGain);
      |     if ~strcmp(f32PropGain_bkup,tmps)
      |       set_param(gcb,'f32PropGain',tmps);
      |     end
      |   end
      |   if isnan(f32IntegGain)
      |     if ~strcmp(f32IntegGain_bkup,'0')
      |       set_param(gcb,'f32IntegGain','0');
      |     end
      |   else
      |     tmps=num2str(f32IntegGain);
      |     if ~strcmp(f32IntegGain_bkup,tmps)
      |       set_param(gcb,'f32IntegGain',tmps);
      |     end
      |   end
      |   if isnan(f32DerivGain)
      |     if ~strcmp(f32DerivGain_bkup,'0')
      |       set_param(gcb,'f32DerivGain','0');
      |     end
      |   else
      |     tmps=num2str(f32DerivGain);
      |     if ~strcmp(f32DerivGain_bkup,tmps)
      |       set_param(gcb,'f32DerivGain',tmps);
      |     end
      |   end
      |   if isnan(f32FiltCoef)
      |     if ~strcmp(f32FiltCoef_bkup,'0')
      |       set_param(gcb,'f32FiltCoef','0');
      |     end
      |   else
      |     tmps=num2str(f32FiltCoef);
      |     if ~strcmp(f32FiltCoef_bkup,tmps)
      |       set_param(gcb,'f32FiltCoef',tmps);
      |     end
      |   end
      |   if isnan(s16PropGainShift)
      |     if ~strcmp(s16PropGainShift_bkup,'0')
      |       set_param(gcb,'s16PropGainShift','0');
      |     end
      |   else
      |     tmps=num2str(s16PropGainShift);
      |     if ~strcmp(s16PropGainShift_bkup,tmps)
      |       set_param(gcb,'s16PropGainShift',tmps);
      |     end
      |   end
      |   if isnan(s16IntegGainShift)
      |     if ~strcmp(s16IntegGainShift_bkup,'0')
      |       set_param(gcb,'s16IntegGainShift','0');
      |     end
      |   else
      |     tmps=num2str(s16IntegGainShift);
      |     if ~strcmp(s16IntegGainShift_bkup,tmps)
      |       set_param(gcb,'s16IntegGainShift',tmps);
      |     end
      |   end
      |   if isnan(s16DerivGainShift)
      |     if ~strcmp(s16DerivGainShift_bkup,'0')
      |       set_param(gcb,'s16DerivGainShift','0');
      |     end
      |   else
      |     tmps=num2str(s16DerivGainShift);
      |     if ~strcmp(s16DerivGainShift_bkup,tmps)
      |       set_param(gcb,'s16DerivGainShift',tmps);
      |     end
      |   end
      |   if isnan(f32LowerLimit)
      |     if ~strcmp(f32LowerLimit_bkup,'0')
      |       set_param(gcb,'f32LowerLimit','0');
      |     end
      |   else
      |     tmps=num2str(f32LowerLimit);
      |     if ~strcmp(f32LowerLimit_bkup,tmps)
      |       set_param(gcb,'f32LowerLimit',tmps);
      |     end
      |   end
      |   if isnan(f32UpperLimit)
      |     if ~strcmp(f32UpperLimit_bkup,'0')
      |       set_param(gcb,'f32UpperLimit','0');
      |     end
      |   else
      |     tmps=num2str(f32UpperLimit);
      |     if ~strcmp(f32UpperLimit_bkup,tmps)
      |       set_param(gcb,'f32UpperLimit',tmps);
      |     end
      |   end
      | end
      mask Callback inscale:
      | autoCalcEn=get_param(gcb,'autoCalcEn');
      | if strcmp(autoCalcEn,'on')
      |   SampleTime=Simulink.data.evalinGlobal(bdroot,get_param(gcb,'SampleTime'));
      |   if (SampleTime==-1)
      |     SampleTime=str2double(get_param(gcb,'SampleTime_1'));
      |   end
      |   f32PropGain_bkup=get_param(gcb,'f32PropGain');
      |   f32IntegGain_bkup=get_param(gcb,'f32IntegGain');
      |   f32DerivGain_bkup=get_param(gcb,'f32DerivGain');
      |   f32FiltCoef_bkup=get_param(gcb,'f32FiltCoef');
      |   s16PropGainShift_bkup=get_param(gcb,'s16PropGainShift');
      |   s16IntegGainShift_bkup=get_param(gcb,'s16IntegGainShift');
      |   s16DerivGainShift_bkup=get_param(gcb,'s16DerivGainShift');
      |   f32LowerLimit_bkup=get_param(gcb,'f32LowerLimit');
      |   f32UpperLimit_bkup=get_param(gcb,'f32UpperLimit');
      |   pgain=Simulink.data.evalinGlobal(bdroot,get_param(gcb,'pgain'));
      |   igain=Simulink.data.evalinGlobal(bdroot,get_param(gcb,'igain'));
      |   dgain=Simulink.data.evalinGlobal(bdroot,get_param(gcb,'dgain'));
      |   filtCoef=Simulink.data.evalinGlobal(bdroot,get_param(gcb,'filtCoef'));
      |   lowerLimit=Simulink.data.evalinGlobal(bdroot,get_param(gcb,'lowerLimit'));
      |   upperLimit=Simulink.data.evalinGlobal(bdroot,get_param(gcb,'upperLimit'));
      |   inscale=Simulink.data.evalinGlobal(bdroot,get_param(gcb,'inscale'));
      |   outscale=Simulink.data.evalinGlobal(bdroot,get_param(gcb,'outscale'));
      |   if (upperLimit<=lowerLimit)
      |     warning('UpperLimit should be greater than LowerLimit.');
      |   end
      |   if (inscale<=0)
      |     warning('E_max must be positive.');
      |   end
      |   if (outscale<=0)
      |     warning('U_max must be positive.');
      |   end
      |   kpf=pgain*inscale/outscale;
      |   s16PropGainShift=ceil(log2(abs(kpf)));
      |   if s16PropGainShift<-31
      |     s16PropGainShift=-31;
      |   end
      |   if s16PropGainShift>31
      |     s16PropGainShift=31;
      |     warning(['Parameter s16PropGainShift of ' gcb ' exceeds the fixed-point range.']);
      |   end
      |   f32PropGain=round(kpf*2^(-s16PropGainShift)*2^31);
      |   if f32PropGain>2^31-1
      |     f32PropGain=2^31-1;
      |     warning(['Parameter f32PropGain of ' gcb ' exceeds the fixed-point range.']);
      |   end
      |   if f32PropGain<-2^31
      |     f32PropGain=-2^31;
      |     warning(['Parameter f32PropGain of ' gcb ' exceeds the fixed-point range.']);
      |   end
      |   kif=igain*SampleTime*0.5*inscale/outscale;
      |   s16IntegGainShift=ceil(log2(abs(kif)));
      |   if s16IntegGainShift<-31
      |     s16IntegGainShift=-31;
      |   end
      |   if s16IntegGainShift>31
      |     s16IntegGainShift=31;
      |     warning(['Parameter s16IntegGainShift of ' gcb ' exceeds the fixed-point range.']);
      |   end
      |   f32IntegGain=round(kif*2^(-s16IntegGainShift)*2^31);
      |   if f32IntegGain>2^31-1
      |     f32IntegGain=2^31-1;
      |     warning(['Parameter f32IntegGain of ' gcb ' exceeds the fixed-point range.']);
      |   end
      |   if f32IntegGain<-2^31
      |     f32IntegGain=-2^31;
      |     warning(['Parameter f32IntegGain of ' gcb ' exceeds the fixed-point range.']);
      |   end
      |   upperLimitf=upperLimit/outscale;
      |   lowerLimitf=lowerLimit/outscale;
      |   f32UpperLimit=round(upperLimitf*2^31);
      |   if f32UpperLimit>2^31-1
      |     f32UpperLimit=2^31-1;
      |     warning(['Parameter f32UpperLimit of ' gcb ' exceeds the fixed-point range.']);
      |   end
      |   if f32UpperLimit<-2^31
      |     f32UpperLimit=-2^31;
      |     warning(['Parameter f32UpperLimit of ' gcb ' exceeds the fixed-point range.']);
      |   end
      |   f32LowerLimit=round(lowerLimitf*2^31);
      |   if f32LowerLimit>2^31-1
      |     f32LowerLimit=2^31-1;
      |     warning(['Parameter f32LowerLimit of ' gcb ' exceeds the fixed-point range.']);
      |   end
      |   if f32LowerLimit<-2^31
      |     f32LowerLimit=-2^31;
      |     warning(['Parameter f32LowerLimit of ' gcb ' exceeds the fixed-point range.']);
      |   end
      |   exparg=-SampleTime*filtCoef;
      |   expconst=exp(exparg);
      |   f32FiltCoef=round(expconst*2^31);
      |   if f32FiltCoef>2^31-1
      |     f32FiltCoef=2^31-1;
      |     warning(['Parameter f32FiltCoef of ' gcb ' exceeds the fixed-point range.']);
      |   end
      |   if f32FiltCoef<-2^31
      |     f32FiltCoef=-2^31;
      |     warning(['Parameter f32FiltCoef of ' gcb ' exceeds the fixed-point range.']);
      |   end
      |   kdf=dgain/SampleTime*(1 - expconst)*inscale/outscale;
      |   s16DerivGainShift=ceil(log2(abs(kpf)));
      |   if s16DerivGainShift<-31
      |     s16DerivGainShift=-31;
      |   end
      |   if s16DerivGainShift>31
      |     s16DerivGainShift=31;
      |     warning(['Parameter s16DerivGainShift of ' gcb ' exceeds the fixed-point range.']);
      |   end
      |   f32DerivGain=round(kpf*2^(-s16DerivGainShift)*2^31);
      |   if f32DerivGain>2^31-1
      |     f32DerivGain=2^31-1;
      |     warning(['Parameter f32DerivGain of ' gcb ' exceeds the fixed-point range.']);
      |   end
      |   if f32DerivGain<-2^31
      |     f32DerivGain=-2^31;
      |     warning(['Parameter f32DerivGain of ' gcb ' exceeds the fixed-point range.']);
      |   end
      |   if isnan(f32PropGain)
      |     if ~strcmp(f32PropGain_bkup,'0')
      |       set_param(gcb,'f32PropGain','0');
      |     end
      |   else
      |     tmps=num2str(f32PropGain);
      |     if ~strcmp(f32PropGain_bkup,tmps)
      |       set_param(gcb,'f32PropGain',tmps);
      |     end
      |   end
      |   if isnan(f32IntegGain)
      |     if ~strcmp(f32IntegGain_bkup,'0')
      |       set_param(gcb,'f32IntegGain','0');
      |     end
      |   else
      |     tmps=num2str(f32IntegGain);
      |     if ~strcmp(f32IntegGain_bkup,tmps)
      |       set_param(gcb,'f32IntegGain',tmps);
      |     end
      |   end
      |   if isnan(f32DerivGain)
      |     if ~strcmp(f32DerivGain_bkup,'0')
      |       set_param(gcb,'f32DerivGain','0');
      |     end
      |   else
      |     tmps=num2str(f32DerivGain);
      |     if ~strcmp(f32DerivGain_bkup,tmps)
      |       set_param(gcb,'f32DerivGain',tmps);
      |     end
      |   end
      |   if isnan(f32FiltCoef)
      |     if ~strcmp(f32FiltCoef_bkup,'0')
      |       set_param(gcb,'f32FiltCoef','0');
      |     end
      |   else
      |     tmps=num2str(f32FiltCoef);
      |     if ~strcmp(f32FiltCoef_bkup,tmps)
      |       set_param(gcb,'f32FiltCoef',tmps);
      |     end
      |   end
      |   if isnan(s16PropGainShift)
      |     if ~strcmp(s16PropGainShift_bkup,'0')
      |       set_param(gcb,'s16PropGainShift','0');
      |     end
      |   else
      |     tmps=num2str(s16PropGainShift);
      |     if ~strcmp(s16PropGainShift_bkup,tmps)
      |       set_param(gcb,'s16PropGainShift',tmps);
      |     end
      |   end
      |   if isnan(s16IntegGainShift)
      |     if ~strcmp(s16IntegGainShift_bkup,'0')
      |       set_param(gcb,'s16IntegGainShift','0');
      |     end
      |   else
      |     tmps=num2str(s16IntegGainShift);
      |     if ~strcmp(s16IntegGainShift_bkup,tmps)
      |       set_param(gcb,'s16IntegGainShift',tmps);
      |     end
      |   end
      |   if isnan(s16DerivGainShift)
      |     if ~strcmp(s16DerivGainShift_bkup,'0')
      |       set_param(gcb,'s16DerivGainShift','0');
      |     end
      |   else
      |     tmps=num2str(s16DerivGainShift);
      |     if ~strcmp(s16DerivGainShift_bkup,tmps)
      |       set_param(gcb,'s16DerivGainShift',tmps);
      |     end
      |   end
      |   if isnan(f32LowerLimit)
      |     if ~strcmp(f32LowerLimit_bkup,'0')
      |       set_param(gcb,'f32LowerLimit','0');
      |     end
      |   else
      |     tmps=num2str(f32LowerLimit);
      |     if ~strcmp(f32LowerLimit_bkup,tmps)
      |       set_param(gcb,'f32LowerLimit',tmps);
      |     end
      |   end
      |   if isnan(f32UpperLimit)
      |     if ~strcmp(f32UpperLimit_bkup,'0')
      |       set_param(gcb,'f32UpperLimit','0');
      |     end
      |   else
      |     tmps=num2str(f32UpperLimit);
      |     if ~strcmp(f32UpperLimit_bkup,tmps)
      |       set_param(gcb,'f32UpperLimit',tmps);
      |     end
      |   end
      | end
      mask Callback outscale:
      | autoCalcEn=get_param(gcb,'autoCalcEn');
      | if strcmp(autoCalcEn,'on')
      |   SampleTime=Simulink.data.evalinGlobal(bdroot,get_param(gcb,'SampleTime'));
      |   if (SampleTime==-1)
      |     SampleTime=str2double(get_param(gcb,'SampleTime_1'));
      |   end
      |   f32PropGain_bkup=get_param(gcb,'f32PropGain');
      |   f32IntegGain_bkup=get_param(gcb,'f32IntegGain');
      |   f32DerivGain_bkup=get_param(gcb,'f32DerivGain');
      |   f32FiltCoef_bkup=get_param(gcb,'f32FiltCoef');
      |   s16PropGainShift_bkup=get_param(gcb,'s16PropGainShift');
      |   s16IntegGainShift_bkup=get_param(gcb,'s16IntegGainShift');
      |   s16DerivGainShift_bkup=get_param(gcb,'s16DerivGainShift');
      |   f32LowerLimit_bkup=get_param(gcb,'f32LowerLimit');
      |   f32UpperLimit_bkup=get_param(gcb,'f32UpperLimit');
      |   pgain=Simulink.data.evalinGlobal(bdroot,get_param(gcb,'pgain'));
      |   igain=Simulink.data.evalinGlobal(bdroot,get_param(gcb,'igain'));
      |   dgain=Simulink.data.evalinGlobal(bdroot,get_param(gcb,'dgain'));
      |   filtCoef=Simulink.data.evalinGlobal(bdroot,get_param(gcb,'filtCoef'));
      |   lowerLimit=Simulink.data.evalinGlobal(bdroot,get_param(gcb,'lowerLimit'));
      |   upperLimit=Simulink.data.evalinGlobal(bdroot,get_param(gcb,'upperLimit'));
      |   inscale=Simulink.data.evalinGlobal(bdroot,get_param(gcb,'inscale'));
      |   outscale=Simulink.data.evalinGlobal(bdroot,get_param(gcb,'outscale'));
      |   if (upperLimit<=lowerLimit)
      |     warning('UpperLimit should be greater than LowerLimit.');
      |   end
      |   if (inscale<=0)
      |     warning('E_max must be positive.');
      |   end
      |   if (outscale<=0)
      |     warning('U_max must be positive.');
      |   end
      |   kpf=pgain*inscale/outscale;
      |   s16PropGainShift=ceil(log2(abs(kpf)));
      |   if s16PropGainShift<-31
      |     s16PropGainShift=-31;
      |   end
      |   if s16PropGainShift>31
      |     s16PropGainShift=31;
      |     warning(['Parameter s16PropGainShift of ' gcb ' exceeds the fixed-point range.']);
      |   end
      |   f32PropGain=round(kpf*2^(-s16PropGainShift)*2^31);
      |   if f32PropGain>2^31-1
      |     f32PropGain=2^31-1;
      |     warning(['Parameter f32PropGain of ' gcb ' exceeds the fixed-point range.']);
      |   end
      |   if f32PropGain<-2^31
      |     f32PropGain=-2^31;
      |     warning(['Parameter f32PropGain of ' gcb ' exceeds the fixed-point range.']);
      |   end
      |   kif=igain*SampleTime*0.5*inscale/outscale;
      |   s16IntegGainShift=ceil(log2(abs(kif)));
      |   if s16IntegGainShift<-31
      |     s16IntegGainShift=-31;
      |   end
      |   if s16IntegGainShift>31
      |     s16IntegGainShift=31;
      |     warning(['Parameter s16IntegGainShift of ' gcb ' exceeds the fixed-point range.']);
      |   end
      |   f32IntegGain=round(kif*2^(-s16IntegGainShift)*2^31);
      |   if f32IntegGain>2^31-1
      |     f32IntegGain=2^31-1;
      |     warning(['Parameter f32IntegGain of ' gcb ' exceeds the fixed-point range.']);
      |   end
      |   if f32IntegGain<-2^31
      |     f32IntegGain=-2^31;
      |     warning(['Parameter f32IntegGain of ' gcb ' exceeds the fixed-point range.']);
      |   end
      |   upperLimitf=upperLimit/outscale;
      |   lowerLimitf=lowerLimit/outscale;
      |   f32UpperLimit=round(upperLimitf*2^31);
      |   if f32UpperLimit>2^31-1
      |     f32UpperLimit=2^31-1;
      |     warning(['Parameter f32UpperLimit of ' gcb ' exceeds the fixed-point range.']);
      |   end
      |   if f32UpperLimit<-2^31
      |     f32UpperLimit=-2^31;
      |     warning(['Parameter f32UpperLimit of ' gcb ' exceeds the fixed-point range.']);
      |   end
      |   f32LowerLimit=round(lowerLimitf*2^31);
      |   if f32LowerLimit>2^31-1
      |     f32LowerLimit=2^31-1;
      |     warning(['Parameter f32LowerLimit of ' gcb ' exceeds the fixed-point range.']);
      |   end
      |   if f32LowerLimit<-2^31
      |     f32LowerLimit=-2^31;
      |     warning(['Parameter f32LowerLimit of ' gcb ' exceeds the fixed-point range.']);
      |   end
      |   exparg=-SampleTime*filtCoef;
      |   expconst=exp(exparg);
      |   f32FiltCoef=round(expconst*2^31);
      |   if f32FiltCoef>2^31-1
      |     f32FiltCoef=2^31-1;
      |     warning(['Parameter f32FiltCoef of ' gcb ' exceeds the fixed-point range.']);
      |   end
      |   if f32FiltCoef<-2^31
      |     f32FiltCoef=-2^31;
      |     warning(['Parameter f32FiltCoef of ' gcb ' exceeds the fixed-point range.']);
      |   end
      |   kdf=dgain/SampleTime*(1 - expconst)*inscale/outscale;
      |   s16DerivGainShift=ceil(log2(abs(kpf)));
      |   if s16DerivGainShift<-31
      |     s16DerivGainShift=-31;
      |   end
      |   if s16DerivGainShift>31
      |     s16DerivGainShift=31;
      |     warning(['Parameter s16DerivGainShift of ' gcb ' exceeds the fixed-point range.']);
      |   end
      |   f32DerivGain=round(kpf*2^(-s16DerivGainShift)*2^31);
      |   if f32DerivGain>2^31-1
      |     f32DerivGain=2^31-1;
      |     warning(['Parameter f32DerivGain of ' gcb ' exceeds the fixed-point range.']);
      |   end
      |   if f32DerivGain<-2^31
      |     f32DerivGain=-2^31;
      |     warning(['Parameter f32DerivGain of ' gcb ' exceeds the fixed-point range.']);
      |   end
      |   if isnan(f32PropGain)
      |     if ~strcmp(f32PropGain_bkup,'0')
      |       set_param(gcb,'f32PropGain','0');
      |     end
      |   else
      |     tmps=num2str(f32PropGain);
      |     if ~strcmp(f32PropGain_bkup,tmps)
      |       set_param(gcb,'f32PropGain',tmps);
      |     end
      |   end
      |   if isnan(f32IntegGain)
      |     if ~strcmp(f32IntegGain_bkup,'0')
      |       set_param(gcb,'f32IntegGain','0');
      |     end
      |   else
      |     tmps=num2str(f32IntegGain);
      |     if ~strcmp(f32IntegGain_bkup,tmps)
      |       set_param(gcb,'f32IntegGain',tmps);
      |     end
      |   end
      |   if isnan(f32DerivGain)
      |     if ~strcmp(f32DerivGain_bkup,'0')
      |       set_param(gcb,'f32DerivGain','0');
      |     end
      |   else
      |     tmps=num2str(f32DerivGain);
      |     if ~strcmp(f32DerivGain_bkup,tmps)
      |       set_param(gcb,'f32DerivGain',tmps);
      |     end
      |   end
      |   if isnan(f32FiltCoef)
      |     if ~strcmp(f32FiltCoef_bkup,'0')
      |       set_param(gcb,'f32FiltCoef','0');
      |     end
      |   else
      |     tmps=num2str(f32FiltCoef);
      |     if ~strcmp(f32FiltCoef_bkup,tmps)
      |       set_param(gcb,'f32FiltCoef',tmps);
      |     end
      |   end
      |   if isnan(s16PropGainShift)
      |     if ~strcmp(s16PropGainShift_bkup,'0')
      |       set_param(gcb,'s16PropGainShift','0');
      |     end
      |   else
      |     tmps=num2str(s16PropGainShift);
      |     if ~strcmp(s16PropGainShift_bkup,tmps)
      |       set_param(gcb,'s16PropGainShift',tmps);
      |     end
      |   end
      |   if isnan(s16IntegGainShift)
      |     if ~strcmp(s16IntegGainShift_bkup,'0')
      |       set_param(gcb,'s16IntegGainShift','0');
      |     end
      |   else
      |     tmps=num2str(s16IntegGainShift);
      |     if ~strcmp(s16IntegGainShift_bkup,tmps)
      |       set_param(gcb,'s16IntegGainShift',tmps);
      |     end
      |   end
      |   if isnan(s16DerivGainShift)
      |     if ~strcmp(s16DerivGainShift_bkup,'0')
      |       set_param(gcb,'s16DerivGainShift','0');
      |     end
      |   else
      |     tmps=num2str(s16DerivGainShift);
      |     if ~strcmp(s16DerivGainShift_bkup,tmps)
      |       set_param(gcb,'s16DerivGainShift',tmps);
      |     end
      |   end
      |   if isnan(f32LowerLimit)
      |     if ~strcmp(f32LowerLimit_bkup,'0')
      |       set_param(gcb,'f32LowerLimit','0');
      |     end
      |   else
      |     tmps=num2str(f32LowerLimit);
      |     if ~strcmp(f32LowerLimit_bkup,tmps)
      |       set_param(gcb,'f32LowerLimit',tmps);
      |     end
      |   end
      |   if isnan(f32UpperLimit)
      |     if ~strcmp(f32UpperLimit_bkup,'0')
      |       set_param(gcb,'f32UpperLimit','0');
      |     end
      |   else
      |     tmps=num2str(f32UpperLimit);
      |     if ~strcmp(f32UpperLimit_bkup,tmps)
      |       set_param(gcb,'f32UpperLimit',tmps);
      |     end
      |   end
      | end
      mask Callback autoCalcEn:
      | maskStr=get_param(gcb,'showStates');
      | if strcmp(maskStr,'Hide (faster execution)')
      |   p=Simulink.Mask.get(gcb);
      |   autoCalcEn=get_param(gcb,'autoCalcEn');
      |   hintText=p.getDialogControl('timeHint');
      |   if strcmp(autoCalcEn,'on')
      |     param=p.getParameter('outscale');
      |     if strcmp(param.Enabled,'off')
      |       SampleTime=Simulink.data.evalinGlobal(bdroot,get_param(gcb,'SampleTime'));
      |       if SampleTime==-1
      |         SampleTime=str2double(get_param(gcb,'SampleTime_1'));
      |         if isnan(SampleTime)
      |           hintText.Prompt=['Note: Implementation parameters cannot be calculated yet because the block''s inherited sample time is unknown. Simulink will update the sample time when you run the simulation.'];
      |         else
      |           hintText.Prompt=['Caution: Implementation parameters depend on inherited sample time. Make sure that the sample time of the block''s inputs corresponds to the sampling period in the target application.'];
      |         end
      |       else
      |         hintText.Prompt='Caution: Implementation parameters depend on the sample time. Make sure that the simulation time step corresponds to the sampling period in the target application.';
      |       end
      |       p=Simulink.Mask.get(gcb);
      |       param=p.getParameter('pgain');
      |       param.set('Enabled','on');
      |       param=p.getParameter('igain');
      |       param.set('Enabled','on');
      |       param=p.getParameter('dgain');
      |       param.set('Enabled','on');
      |       param=p.getParameter('filtCoef');
      |       param.set('Enabled','on');
      |       param=p.getParameter('lowerLimit');
      |       param.set('Enabled','on');
      |       param=p.getParameter('upperLimit');
      |       param.set('Enabled','on');
      |       param=p.getParameter('inscale');
      |       param.set('Enabled','on');
      |       param=p.getParameter('outscale');
      |       param.set('Enabled','on');
      |     else
      |       SampleTime=Simulink.data.evalinGlobal(bdroot,get_param(gcb,'SampleTime'));
      |       if SampleTime==-1
      |         SampleTime=str2double(get_param(gcb,'SampleTime_1'));
      |       end
      |     end
      |     f32PropGain_bkup=get_param(gcb,'f32PropGain');
      |     f32IntegGain_bkup=get_param(gcb,'f32IntegGain');
      |     f32DerivGain_bkup=get_param(gcb,'f32DerivGain');
      |     f32FiltCoef_bkup=get_param(gcb,'f32FiltCoef');
      |     s16PropGainShift_bkup=get_param(gcb,'s16PropGainShift');
      |     s16IntegGainShift_bkup=get_param(gcb,'s16IntegGainShift');
      |     s16DerivGainShift_bkup=get_param(gcb,'s16DerivGainShift');
      |     f32LowerLimit_bkup=get_param(gcb,'f32LowerLimit');
      |     f32UpperLimit_bkup=get_param(gcb,'f32UpperLimit');
      |     pgain=Simulink.data.evalinGlobal(bdroot,get_param(gcb,'pgain'));
      |     igain=Simulink.data.evalinGlobal(bdroot,get_param(gcb,'igain'));
      |     dgain=Simulink.data.evalinGlobal(bdroot,get_param(gcb,'dgain'));
      |     filtCoef=Simulink.data.evalinGlobal(bdroot,get_param(gcb,'filtCoef'));
      |     lowerLimit=Simulink.data.evalinGlobal(bdroot,get_param(gcb,'lowerLimit'));
      |     upperLimit=Simulink.data.evalinGlobal(bdroot,get_param(gcb,'upperLimit'));
      |     inscale=Simulink.data.evalinGlobal(bdroot,get_param(gcb,'inscale'));
      |     outscale=Simulink.data.evalinGlobal(bdroot,get_param(gcb,'outscale'));
      |     if (upperLimit<=lowerLimit)
      |       warning('UpperLimit should be greater than LowerLimit.');
      |     end
      |     if (inscale<=0)
      |       warning('E_max must be positive.');
      |     end
      |     if (outscale<=0)
      |       warning('U_max must be positive.');
      |     end
      |     kpf=pgain*inscale/outscale;
      |     s16PropGainShift=ceil(log2(abs(kpf)));
      |     if s16PropGainShift<-31
      |       s16PropGainShift=-31;
      |     end
      |     if s16PropGainShift>31
      |       s16PropGainShift=31;
      |       warning(['Parameter s16PropGainShift of ' gcb ' exceeds the fixed-point range.']);
      |     end
      |     f32PropGain=round(kpf*2^(-s16PropGainShift)*2^31);
      |     if f32PropGain>2^31-1
      |       f32PropGain=2^31-1;
      |       warning(['Parameter f32PropGain of ' gcb ' exceeds the fixed-point range.']);
      |     end
      |     if f32PropGain<-2^31
      |       f32PropGain=-2^31;
      |       warning(['Parameter f32PropGain of ' gcb ' exceeds the fixed-point range.']);
      |     end
      |     kif=igain*SampleTime*0.5*inscale/outscale;
      |     s16IntegGainShift=ceil(log2(abs(kif)));
      |     if s16IntegGainShift<-31
      |       s16IntegGainShift=-31;
      |     end
      |     if s16IntegGainShift>31
      |       s16IntegGainShift=31;
      |       warning(['Parameter s16IntegGainShift of ' gcb ' exceeds the fixed-point range.']);
      |     end
      |     f32IntegGain=round(kif*2^(-s16IntegGainShift)*2^31);
      |     if f32IntegGain>2^31-1
      |       f32IntegGain=2^31-1;
      |       warning(['Parameter f32IntegGain of ' gcb ' exceeds the fixed-point range.']);
      |     end
      |     if f32IntegGain<-2^31
      |       f32IntegGain=-2^31;
      |       warning(['Parameter f32IntegGain of ' gcb ' exceeds the fixed-point range.']);
      |     end
      |     upperLimitf=upperLimit/outscale;
      |     lowerLimitf=lowerLimit/outscale;
      |     f32UpperLimit=round(upperLimitf*2^31);
      |     if f32UpperLimit>2^31-1
      |       f32UpperLimit=2^31-1;
      |       warning(['Parameter f32UpperLimit of ' gcb ' exceeds the fixed-point range.']);
      |     end
      |     if f32UpperLimit<-2^31
      |       f32UpperLimit=-2^31;
      |       warning(['Parameter f32UpperLimit of ' gcb ' exceeds the fixed-point range.']);
      |     end
      |     f32LowerLimit=round(lowerLimitf*2^31);
      |     if f32LowerLimit>2^31-1
      |       f32LowerLimit=2^31-1;
      |       warning(['Parameter f32LowerLimit of ' gcb ' exceeds the fixed-point range.']);
      |     end
      |     if f32LowerLimit<-2^31
      |       f32LowerLimit=-2^31;
      |       warning(['Parameter f32LowerLimit of ' gcb ' exceeds the fixed-point range.']);
      |     end
      |     exparg=-SampleTime*filtCoef;
      |     expconst=exp(exparg);
      |     f32FiltCoef=round(expconst*2^31);
      |     if f32FiltCoef>2^31-1
      |       f32FiltCoef=2^31-1;
      |       warning(['Parameter f32FiltCoef of ' gcb ' exceeds the fixed-point range.']);
      |     end
      |     if f32FiltCoef<-2^31
      |       f32FiltCoef=-2^31;
      |       warning(['Parameter f32FiltCoef of ' gcb ' exceeds the fixed-point range.']);
      |     end
      |     kdf=dgain/SampleTime*(1 - expconst)*inscale/outscale;
      |     s16DerivGainShift=ceil(log2(abs(kpf)));
      |     if s16DerivGainShift<-31
      |       s16DerivGainShift=-31;
      |     end
      |     if s16DerivGainShift>31
      |       s16DerivGainShift=31;
      |       warning(['Parameter s16DerivGainShift of ' gcb ' exceeds the fixed-point range.']);
      |     end
      |     f32DerivGain=round(kpf*2^(-s16DerivGainShift)*2^31);
      |     if f32DerivGain>2^31-1
      |       f32DerivGain=2^31-1;
      |       warning(['Parameter f32DerivGain of ' gcb ' exceeds the fixed-point range.']);
      |     end
      |     if f32DerivGain<-2^31
      |       f32DerivGain=-2^31;
      |       warning(['Parameter f32DerivGain of ' gcb ' exceeds the fixed-point range.']);
      |     end
      |     if isnan(f32PropGain)
      |       if ~strcmp(f32PropGain_bkup,'0')
      |         set_param(gcb,'f32PropGain','0');
      |       end
      |     else
      |       tmps=num2str(f32PropGain);
      |       if ~strcmp(f32PropGain_bkup,tmps)
      |         set_param(gcb,'f32PropGain',tmps);
      |       end
      |     end
      |     if isnan(f32IntegGain)
      |       if ~strcmp(f32IntegGain_bkup,'0')
      |         set_param(gcb,'f32IntegGain','0');
      |       end
      |     else
      |       tmps=num2str(f32IntegGain);
      |       if ~strcmp(f32IntegGain_bkup,tmps)
      |         set_param(gcb,'f32IntegGain',tmps);
      |       end
      |     end
      |     if isnan(f32DerivGain)
      |       if ~strcmp(f32DerivGain_bkup,'0')
      |         set_param(gcb,'f32DerivGain','0');
      |       end
      |     else
      |       tmps=num2str(f32DerivGain);
      |       if ~strcmp(f32DerivGain_bkup,tmps)
      |         set_param(gcb,'f32DerivGain',tmps);
      |       end
      |     end
      |     if isnan(f32FiltCoef)
      |       if ~strcmp(f32FiltCoef_bkup,'0')
      |         set_param(gcb,'f32FiltCoef','0');
      |       end
      |     else
      |       tmps=num2str(f32FiltCoef);
      |       if ~strcmp(f32FiltCoef_bkup,tmps)
      |         set_param(gcb,'f32FiltCoef',tmps);
      |       end
      |     end
      |     if isnan(s16PropGainShift)
      |       if ~strcmp(s16PropGainShift_bkup,'0')
      |         set_param(gcb,'s16PropGainShift','0');
      |       end
      |     else
      |       tmps=num2str(s16PropGainShift);
      |       if ~strcmp(s16PropGainShift_bkup,tmps)
      |         set_param(gcb,'s16PropGainShift',tmps);
      |       end
      |     end
      |     if isnan(s16IntegGainShift)
      |       if ~strcmp(s16IntegGainShift_bkup,'0')
      |         set_param(gcb,'s16IntegGainShift','0');
      |       end
      |     else
      |       tmps=num2str(s16IntegGainShift);
      |       if ~strcmp(s16IntegGainShift_bkup,tmps)
      |         set_param(gcb,'s16IntegGainShift',tmps);
      |       end
      |     end
      |     if isnan(s16DerivGainShift)
      |       if ~strcmp(s16DerivGainShift_bkup,'0')
      |         set_param(gcb,'s16DerivGainShift','0');
      |       end
      |     else
      |       tmps=num2str(s16DerivGainShift);
      |       if ~strcmp(s16DerivGainShift_bkup,tmps)
      |         set_param(gcb,'s16DerivGainShift',tmps);
      |       end
      |     end
      |     if isnan(f32LowerLimit)
      |       if ~strcmp(f32LowerLimit_bkup,'0')
      |         set_param(gcb,'f32LowerLimit','0');
      |       end
      |     else
      |       tmps=num2str(f32LowerLimit);
      |       if ~strcmp(f32LowerLimit_bkup,tmps)
      |         set_param(gcb,'f32LowerLimit',tmps);
      |       end
      |     end
      |     if isnan(f32UpperLimit)
      |       if ~strcmp(f32UpperLimit_bkup,'0')
      |         set_param(gcb,'f32UpperLimit','0');
      |       end
      |     else
      |       tmps=num2str(f32UpperLimit);
      |       if ~strcmp(f32UpperLimit_bkup,tmps)
      |         set_param(gcb,'f32UpperLimit',tmps);
      |       end
      |     end
      |   else
      |     param=p.getParameter('outscale');
      |     if strcmp(param.Enabled,'on')
      |       hintText.Prompt='Caution: Implementation parameters are fixed.';
      |       p=Simulink.Mask.get(gcb);
      |       param=p.getParameter('pgain');
      |       param.set('Enabled','off');
      |       param=p.getParameter('igain');
      |       param.set('Enabled','off');
      |       param=p.getParameter('dgain');
      |       param.set('Enabled','off');
      |       param=p.getParameter('filtCoef');
      |       param.set('Enabled','off');
      |       param=p.getParameter('lowerLimit');
      |       param.set('Enabled','off');
      |       param=p.getParameter('upperLimit');
      |       param.set('Enabled','off');
      |       param=p.getParameter('inscale');
      |       param.set('Enabled','off');
      |       param=p.getParameter('outscale');
      |       param.set('Enabled','off');
      |     end
      |   end
      | end
      mask DialogControl CompBut Prompt: Recalculate sample times
      mask DialogControl CompBut Tooltip: Simulink updates the sample times of all blocks when the simulation is run. This button will update the sample times now.
      mask DialogControl CompBut Callback:
      | btn=questdlg('This will apply all changes in all open dialog boxes and update the schematic. Do you want to proceed?','Apply all changes','Continue','Cancel','Continue');
      | if strcmp(btn,'Continue')
      |   dlgs=DAStudio.ToolRoot.getOpenDialogs;
      |   for i=1:length(dlgs)
      |     dlgs(i).apply;
      |   end
      |   try
      |     SampleTime_1=str2double(get_param(gcb,'SampleTime_1'));
      |     ts=Simulink.Block.getSampleTimes(gcb);
      |     ts=ts(1).Value(1);
      |     if (SampleTime_1 ~= ts)
      |       SampleTime_1=ts;
      |       set_param(gcb,'SampleTime_1',num2str(ts));
      |       autoCalcEn=get_param(gcb,'autoCalcEn');
      |       if strcmp(autoCalcEn,'on')
      |         SampleTime=Simulink.data.evalinGlobal(bdroot,get_param(gcb,'SampleTime'));
      |         p=Simulink.Mask.get(gcb);
      |         hintText=p.getDialogControl('timeHint');
      |         if SampleTime==-1
      |           SampleTime=SampleTime_1;
      |           hintText.Prompt='Caution: Implementation parameters depend on inherited sample time. Make sure that the sample time of the block''s inputs corresponds to the sampling period in the target application.';
      |         else
      |           hintText.Prompt='Caution: Implementation parameters depend on the sample time. Make sure that the simulation time step corresponds to the sampling period in the target application.';
      |         end
      |         f32PropGain_bkup=get_param(gcb,'f32PropGain');
      |         f32IntegGain_bkup=get_param(gcb,'f32IntegGain');
      |         f32DerivGain_bkup=get_param(gcb,'f32DerivGain');
      |         f32FiltCoef_bkup=get_param(gcb,'f32FiltCoef');
      |         s16PropGainShift_bkup=get_param(gcb,'s16PropGainShift');
      |         s16IntegGainShift_bkup=get_param(gcb,'s16IntegGainShift');
      |         s16DerivGainShift_bkup=get_param(gcb,'s16DerivGainShift');
      |         f32LowerLimit_bkup=get_param(gcb,'f32LowerLimit');
      |         f32UpperLimit_bkup=get_param(gcb,'f32UpperLimit');
      |         pgain=Simulink.data.evalinGlobal(bdroot,get_param(gcb,'pgain'));
      |         igain=Simulink.data.evalinGlobal(bdroot,get_param(gcb,'igain'));
      |         dgain=Simulink.data.evalinGlobal(bdroot,get_param(gcb,'dgain'));
      |         filtCoef=Simulink.data.evalinGlobal(bdroot,get_param(gcb,'filtCoef'));
      |         lowerLimit=Simulink.data.evalinGlobal(bdroot,get_param(gcb,'lowerLimit'));
      |         upperLimit=Simulink.data.evalinGlobal(bdroot,get_param(gcb,'upperLimit'));
      |         inscale=Simulink.data.evalinGlobal(bdroot,get_param(gcb,'inscale'));
      |         outscale=Simulink.data.evalinGlobal(bdroot,get_param(gcb,'outscale'));
      |         if (upperLimit<=lowerLimit)
      |           warning('UpperLimit should be greater than LowerLimit.');
      |         end
      |         if (inscale<=0)
      |           warning('E_max must be positive.');
      |         end
      |         if (outscale<=0)
      |           warning('U_max must be positive.');
      |         end
      |         kpf=pgain*inscale/outscale;
      |         s16PropGainShift=ceil(log2(abs(kpf)));
      |         if s16PropGainShift<-31
      |           s16PropGainShift=-31;
      |         end
      |         if s16PropGainShift>31
      |           s16PropGainShift=31;
      |           warning(['Parameter s16PropGainShift of ' gcb ' exceeds the fixed-point range.']);
      |         end
      |         f32PropGain=round(kpf*2^(-s16PropGainShift)*2^31);
      |         if f32PropGain>2^31-1
      |           f32PropGain=2^31-1;
      |           warning(['Parameter f32PropGain of ' gcb ' exceeds the fixed-point range.']);
      |         end
      |         if f32PropGain<-2^31
      |           f32PropGain=-2^31;
      |           warning(['Parameter f32PropGain of ' gcb ' exceeds the fixed-point range.']);
      |         end
      |         kif=igain*SampleTime*0.5*inscale/outscale;
      |         s16IntegGainShift=ceil(log2(abs(kif)));
      |         if s16IntegGainShift<-31
      |           s16IntegGainShift=-31;
      |         end
      |         if s16IntegGainShift>31
      |           s16IntegGainShift=31;
      |           warning(['Parameter s16IntegGainShift of ' gcb ' exceeds the fixed-point range.']);
      |         end
      |         f32IntegGain=round(kif*2^(-s16IntegGainShift)*2^31);
      |         if f32IntegGain>2^31-1
      |           f32IntegGain=2^31-1;
      |           warning(['Parameter f32IntegGain of ' gcb ' exceeds the fixed-point range.']);
      |         end
      |         if f32IntegGain<-2^31
      |           f32IntegGain=-2^31;
      |           warning(['Parameter f32IntegGain of ' gcb ' exceeds the fixed-point range.']);
      |         end
      |         upperLimitf=upperLimit/outscale;
      |         lowerLimitf=lowerLimit/outscale;
      |         f32UpperLimit=round(upperLimitf*2^31);
      |         if f32UpperLimit>2^31-1
      |           f32UpperLimit=2^31-1;
      |           warning(['Parameter f32UpperLimit of ' gcb ' exceeds the fixed-point range.']);
      |         end
      |         if f32UpperLimit<-2^31
      |           f32UpperLimit=-2^31;
      |           warning(['Parameter f32UpperLimit of ' gcb ' exceeds the fixed-point range.']);
      |         end
      |         f32LowerLimit=round(lowerLimitf*2^31);
      |         if f32LowerLimit>2^31-1
      |           f32LowerLimit=2^31-1;
      |           warning(['Parameter f32LowerLimit of ' gcb ' exceeds the fixed-point range.']);
      |         end
      |         if f32LowerLimit<-2^31
      |           f32LowerLimit=-2^31;
      |           warning(['Parameter f32LowerLimit of ' gcb ' exceeds the fixed-point range.']);
      |         end
      |         exparg=-SampleTime*filtCoef;
      |         expconst=exp(exparg);
      |         f32FiltCoef=round(expconst*2^31);
      |         if f32FiltCoef>2^31-1
      |           f32FiltCoef=2^31-1;
      |           warning(['Parameter f32FiltCoef of ' gcb ' exceeds the fixed-point range.']);
      |         end
      |         if f32FiltCoef<-2^31
      |           f32FiltCoef=-2^31;
      |           warning(['Parameter f32FiltCoef of ' gcb ' exceeds the fixed-point range.']);
      |         end
      |         kdf=dgain/SampleTime*(1 - expconst)*inscale/outscale;
      |         s16DerivGainShift=ceil(log2(abs(kpf)));
      |         if s16DerivGainShift<-31
      |           s16DerivGainShift=-31;
      |         end
      |         if s16DerivGainShift>31
      |           s16DerivGainShift=31;
      |           warning(['Parameter s16DerivGainShift of ' gcb ' exceeds the fixed-point range.']);
      |         end
      |         f32DerivGain=round(kpf*2^(-s16DerivGainShift)*2^31);
      |         if f32DerivGain>2^31-1
      |           f32DerivGain=2^31-1;
      |           warning(['Parameter f32DerivGain of ' gcb ' exceeds the fixed-point range.']);
      |         end
      |         if f32DerivGain<-2^31
      |           f32DerivGain=-2^31;
      |           warning(['Parameter f32DerivGain of ' gcb ' exceeds the fixed-point range.']);
      |         end
      |         if isnan(f32PropGain)
      |           if ~strcmp(f32PropGain_bkup,'0')
      |             set_param(gcb,'f32PropGain','0');
      |           end
      |         else
      |           tmps=num2str(f32PropGain);
      |           if ~strcmp(f32PropGain_bkup,tmps)
      |             set_param(gcb,'f32PropGain',tmps);
      |           end
      |         end
      |         if isnan(f32IntegGain)
      |           if ~strcmp(f32IntegGain_bkup,'0')
      |             set_param(gcb,'f32IntegGain','0');
      |           end
      |         else
      |           tmps=num2str(f32IntegGain);
      |           if ~strcmp(f32IntegGain_bkup,tmps)
      |             set_param(gcb,'f32IntegGain',tmps);
      |           end
      |         end
      |         if isnan(f32DerivGain)
      |           if ~strcmp(f32DerivGain_bkup,'0')
      |             set_param(gcb,'f32DerivGain','0');
      |           end
      |         else
      |           tmps=num2str(f32DerivGain);
      |           if ~strcmp(f32DerivGain_bkup,tmps)
      |             set_param(gcb,'f32DerivGain',tmps);
      |           end
      |         end
      |         if isnan(f32FiltCoef)
      |           if ~strcmp(f32FiltCoef_bkup,'0')
      |             set_param(gcb,'f32FiltCoef','0');
      |           end
      |         else
      |           tmps=num2str(f32FiltCoef);
      |           if ~strcmp(f32FiltCoef_bkup,tmps)
      |             set_param(gcb,'f32FiltCoef',tmps);
      |           end
      |         end
      |         if isnan(s16PropGainShift)
      |           if ~strcmp(s16PropGainShift_bkup,'0')
      |             set_param(gcb,'s16PropGainShift','0');
      |           end
      |         else
      |           tmps=num2str(s16PropGainShift);
      |           if ~strcmp(s16PropGainShift_bkup,tmps)
      |             set_param(gcb,'s16PropGainShift',tmps);
      |           end
      |         end
      |         if isnan(s16IntegGainShift)
      |           if ~strcmp(s16IntegGainShift_bkup,'0')
      |             set_param(gcb,'s16IntegGainShift','0');
      |           end
      |         else
      |           tmps=num2str(s16IntegGainShift);
      |           if ~strcmp(s16IntegGainShift_bkup,tmps)
      |             set_param(gcb,'s16IntegGainShift',tmps);
      |           end
      |         end
      |         if isnan(s16DerivGainShift)
      |           if ~strcmp(s16DerivGainShift_bkup,'0')
      |             set_param(gcb,'s16DerivGainShift','0');
      |           end
      |         else
      |           tmps=num2str(s16DerivGainShift);
      |           if ~strcmp(s16DerivGainShift_bkup,tmps)
      |             set_param(gcb,'s16DerivGainShift',tmps);
      |           end
      |         end
      |         if isnan(f32LowerLimit)
      |           if ~strcmp(f32LowerLimit_bkup,'0')
      |             set_param(gcb,'f32LowerLimit','0');
      |           end
      |         else
      |           tmps=num2str(f32LowerLimit);
      |           if ~strcmp(f32LowerLimit_bkup,tmps)
      |             set_param(gcb,'f32LowerLimit',tmps);
      |           end
      |         end
      |         if isnan(f32UpperLimit)
      |           if ~strcmp(f32UpperLimit_bkup,'0')
      |             set_param(gcb,'f32UpperLimit','0');
      |           end
      |         else
      |           tmps=num2str(f32UpperLimit);
      |           if ~strcmp(f32UpperLimit_bkup,tmps)
      |             set_param(gcb,'f32UpperLimit',tmps);
      |           end
      |         end
      |       end
      |     end
      |   catch
      |    warning(['Sample time cannot be calculated for the block ' gcb])
      |   end
      | end
      mask DialogControl timeHint Prompt: Note: Implementation parameters cannot be calculated yet because the block's inherited sample time is unknown. Simulink will update the sample time when you run the simulation.
      mask Display:
      | color('black');
      | pos = get_param(gcb, 'Position');
      | width = pos(3) - pos(1);
      | height = pos(4) - pos(2);
      | tX=width/2;
      | tY=height - 25;
      | color('black');
      | text(tX,tY, 'GFLIB_ControllerPIDpAW_F32', 'horizontalAlignment', 'center');
      | if showStates == 2
      |   color('red');
      |   text(tX,tY - 20, ['debugging mode' char(13) char(10) '(limited performance)'], 'horizontalAlignment', 'center');
      | end
  GFLIB_ControllerPIpAW_F32 : Subsystem  StartFcn=|  TreatAsAtomicUnit=on  mask(GFLIB_ControllerPIpAW_F32){showStates=Hide (faster execution), resetStatesEnable=Pre-set according to the first set of inputs after reset, SampleTime=-1, pgain=5, igain=0.5, lowerLimit=-10, upperLimit=9.999999995343387, inscale=10, outscale=10, autoCalcEn=on, f32PropGain=0, f32IntegGain=0, s16PropGainShift=0, s16IntegGainShift=0, f32LowerLimit=0, f32UpperLimit=0, SampleTime_1=NaN}
      | ts=get_param(gcb,'CompiledSampleTime');
      | if iscell(ts)
      |   ts=ts{1};
      |   if iscell(ts)
      |     ts=ts{1};
      |   end
      | end
      | ts=ts(1);
      | set_param(gcb,'SampleTime_1',num2str(ts));
      | p=Simulink.Mask.get(gcb);
      | hintText=p.getDialogControl('timeHint');
      | SampleTime=Simulink.data.evalinGlobal(bdroot,get_param(gcb,'SampleTime'));
      | p=Simulink.Mask.get(gcb);
      | autoCalcEn=get_param(gcb,'autoCalcEn');
      | if strcmp(autoCalcEn,'on')
      |   if SampleTime==-1
      |     hintText.Prompt='Caution: Implementation parameters depend on inherited sample time. Make sure that the sample time of the block''s inputs corresponds to the sampling period in the target application.';
      |   else
      |     hintText.Prompt='Caution: Implementation parameters depend on the sample time. Make sure that the simulation time step corresponds to the sampling period in the target application.';
      |   end
      |   SampleTime=ts;
      |   f32PropGain_bkup=get_param(gcb,'f32PropGain');
      |   f32IntegGain_bkup=get_param(gcb,'f32IntegGain');
      |   s16PropGainShift_bkup=get_param(gcb,'s16PropGainShift');
      |   s16IntegGainShift_bkup=get_param(gcb,'s16IntegGainShift');
      |   f32LowerLimit_bkup=get_param(gcb,'f32LowerLimit');
      |   f32UpperLimit_bkup=get_param(gcb,'f32UpperLimit');
      |   pgain=Simulink.data.evalinGlobal(bdroot,get_param(gcb,'pgain'));
      |   igain=Simulink.data.evalinGlobal(bdroot,get_param(gcb,'igain'));
      |   lowerLimit=Simulink.data.evalinGlobal(bdroot,get_param(gcb,'lowerLimit'));
      |   upperLimit=Simulink.data.evalinGlobal(bdroot,get_param(gcb,'upperLimit'));
      |   inscale=Simulink.data.evalinGlobal(bdroot,get_param(gcb,'inscale'));
      |   outscale=Simulink.data.evalinGlobal(bdroot,get_param(gcb,'outscale'));
      |   if (upperLimit<=lowerLimit)
      |     warning('UpperLimit should be greater than LowerLimit.');
      |   end
      |   if (inscale<=0)
      |     warning('E_max must be positive.');
      |   end
      |   if (outscale<=0)
      |     warning('U_max must be positive.');
      |   end
      |   kpf=pgain*inscale/outscale;
      |   s16PropGainShift=ceil(log2(abs(kpf)));
      |   if s16PropGainShift<-31
      |     s16PropGainShift=-31;
      |   end
      |   if s16PropGainShift>31
      |     s16PropGainShift=31;
      |     warning(['Parameter s16PropGainShift of ' gcb ' exceeds the fixed-point range.']);
      |   end
      |   f32PropGain=round(kpf*2^(-s16PropGainShift)*2^31);
      |   if f32PropGain>2^31-1
      |     f32PropGain=2^31-1;
      |     warning(['Parameter f32PropGain of ' gcb ' exceeds the fixed-point range.']);
      |   end
      |   if f32PropGain<-2^31
      |     f32PropGain=-2^31;
      |     warning(['Parameter f32PropGain of ' gcb ' exceeds the fixed-point range.']);
      |   end
      |   kif=igain*SampleTime*0.5*inscale/outscale;
      |   s16IntegGainShift=ceil(log2(abs(kif)));
      |   if s16IntegGainShift<-31
      |     s16IntegGainShift=-31;
      |   end
      |   if s16IntegGainShift>31
      |     s16IntegGainShift=31;
      |     warning(['Parameter s16IntegGainShift of ' gcb ' exceeds the fixed-point range.']);
      |   end
      |   f32IntegGain=round(kif*2^(-s16IntegGainShift)*2^31);
      |   if f32IntegGain>2^31-1
      |     f32IntegGain=2^31-1;
      |     warning(['Parameter f32IntegGain of ' gcb ' exceeds the fixed-point range.']);
      |   end
      |   if f32IntegGain<-2^31
      |     f32IntegGain=-2^31;
      |     warning(['Parameter f32IntegGain of ' gcb ' exceeds the fixed-point range.']);
      |   end
      |   upperLimitf=upperLimit/outscale;
      |   lowerLimitf=lowerLimit/outscale;
      |   f32UpperLimit=round(upperLimitf*2^31);
      |   if f32UpperLimit>2^31-1
      |     f32UpperLimit=2^31-1;
      |     warning(['Parameter f32UpperLimit of ' gcb ' exceeds the fixed-point range.']);
      |   end
      |   if f32UpperLimit<-2^31
      |     f32UpperLimit=-2^31;
      |     warning(['Parameter f32UpperLimit of ' gcb ' exceeds the fixed-point range.']);
      |   end
      |   f32LowerLimit=round(lowerLimitf*2^31);
      |   if f32LowerLimit>2^31-1
      |     f32LowerLimit=2^31-1;
      |     warning(['Parameter f32LowerLimit of ' gcb ' exceeds the fixed-point range.']);
      |   end
      |   if f32LowerLimit<-2^31
      |     f32LowerLimit=-2^31;
      |     warning(['Parameter f32LowerLimit of ' gcb ' exceeds the fixed-point range.']);
      |   end
      |   if isnan(f32PropGain)
      |     if ~strcmp(f32PropGain_bkup,'0')
      |       set_param(gcb,'f32PropGain','0');
      |     end
      |   else
      |     tmps=num2str(f32PropGain);
      |     if ~strcmp(f32PropGain_bkup,tmps)
      |       set_param(gcb,'f32PropGain',tmps);
      |     end
      |   end
      |   if isnan(f32IntegGain)
      |     if ~strcmp(f32IntegGain_bkup,'0')
      |       set_param(gcb,'f32IntegGain','0');
      |     end
      |   else
      |     tmps=num2str(f32IntegGain);
      |     if ~strcmp(f32IntegGain_bkup,tmps)
      |       set_param(gcb,'f32IntegGain',tmps);
      |     end
      |   end
      |   if isnan(s16PropGainShift)
      |     if ~strcmp(s16PropGainShift_bkup,'0')
      |       set_param(gcb,'s16PropGainShift','0');
      |     end
      |   else
      |     tmps=num2str(s16PropGainShift);
      |     if ~strcmp(s16PropGainShift_bkup,tmps)
      |       set_param(gcb,'s16PropGainShift',tmps);
      |     end
      |   end
      |   if isnan(s16IntegGainShift)
      |     if ~strcmp(s16IntegGainShift_bkup,'0')
      |       set_param(gcb,'s16IntegGainShift','0');
      |     end
      |   else
      |     tmps=num2str(s16IntegGainShift);
      |     if ~strcmp(s16IntegGainShift_bkup,tmps)
      |       set_param(gcb,'s16IntegGainShift',tmps);
      |     end
      |   end
      |   if isnan(f32LowerLimit)
      |     if ~strcmp(f32LowerLimit_bkup,'0')
      |       set_param(gcb,'f32LowerLimit','0');
      |     end
      |   else
      |     tmps=num2str(f32LowerLimit);
      |     if ~strcmp(f32LowerLimit_bkup,tmps)
      |       set_param(gcb,'f32LowerLimit',tmps);
      |     end
      |   end
      |   if isnan(f32UpperLimit)
      |     if ~strcmp(f32UpperLimit_bkup,'0')
      |       set_param(gcb,'f32UpperLimit','0');
      |     end
      |   else
      |     tmps=num2str(f32UpperLimit);
      |     if ~strcmp(f32UpperLimit_bkup,tmps)
      |       set_param(gcb,'f32UpperLimit',tmps);
      |     end
      |   end
      | end
